simulink model "SingleStreamSSR"  (R2020a)
settings: Solver=VariableStepAuto  StartTime=0.0  StopTime=4096  RelTol=1e-3
PreLoadFcn:
  | xmcCheckSlxPath(bdroot)
  | SSR4_init
undefined symbols (not defined in the file): FIR_MultiKernel_cin, FIR_MultiKernel_cincout, FIR_MultiKernel_cout, N, SHIFT_ACC, SingleStream, Taps, xc7vx485tffg1157
libraries: ModelComposer x37, dspsrcs4 x1, simulink x1
(part 2 of 3)

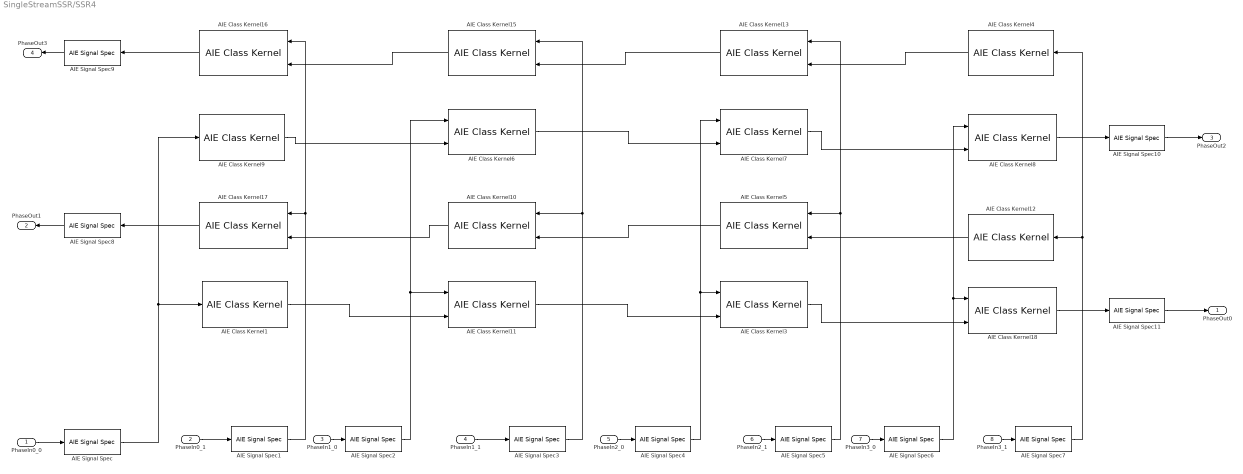
== system SingleStreamSSR/SSR4 ==
  PhaseIn0_0 : Inport
  PhaseIn0_1 : Inport  Port=2
  PhaseIn1_0 : Inport  Port=3
  PhaseIn1_1 : Inport  Port=4
  PhaseIn2_0 : Inport  Port=5
  PhaseIn2_1 : Inport  Port=6
  PhaseIn3_0 : Inport  Port=7
  PhaseIn3_1 : Inport  Port=8
  AIE Class Kernel1 : ModelComposer/AIE Class Kernel  KernelAllAttrs=|  PortNames={'sin'; 'cout'}  PortSerializedTypes={'{P{Tinput_stream{1{t{Scint16}}}}}'; '{P{Toutput_stream{1{t{Scacc48_t}}}}}'}  PortWindowSizes={0.000000000000000000e+00; 0.000000000000000000e+00}  PortWindowMargins={0.000000000000000000e+00; 0.000000000000000000e+00}  PortSynchronicities={'auto'; 'auto'}  PortSignalSizes={0.000000000000000000e+00; 4.000000000000000000e+00}  ClassTemplateSpecKind=implicit  ClassTemplateParamNames={'NSamples'; 'ShiftAcc'}  ClassTemplateParamKinds={'nontype'; 'nontype'}  ClassTemplateParamTypes={'int'; 'int'}  ClassTemplateParamValues={'512', '15'}  ClassCtorParamNames={'taps'; 'Delay'}  ClassCtorParamSerializedTypes={'{R{Q1{C{Scint16}8}}}'; '{Q1{Bi32}}'}  ClassCtorParamValues={'[-54-21i -121-233i 102-525i 237-96i 8773-2748i 1454+497i 342+439i 14+121i]', '0'}  ClassIndex=1  ClassCtorIndex=1  ClassTabVisible=on  ClassTemplateParamsVisible=on  ClassCtorDeclVisible=on  ClassCtorParamsVisible=on  FunctionTabVisible=on  FunctionDecl=|  PortAttrs={ 'input', 'sin', 'input_stream_cint16 *', '', '', '', ''; 'output', 'cout', 'output_stream< cacc48_t > *', '', '', '', 'N' }  PortAttrsEnables={'off', 'off', 'off', 'off', 'off', 'off', 'off';'off', 'off', 'off', 'off', 'off', 'off', 'on'}  SampleTime=-1  ClassDeclTypeOptions=|  ClassDecl=|  ClassTemplateParams={ 'NSamples', 'int', 'BURST_LENGTH'; 'ShiftAcc', 'int', 'SHIFT_ACC' }  ClassTemplateParamsEnables={'off', 'off', 'on';'off', 'off', 'on'}  ClassCtorDeclTypeOptions=C[1 1]@t70@FIR_MultiKernel_cout(cint16 const ( & taps ) [ 8 ], int32 const Delay)  ClassCtorDecl=FIR_MultiKernel_cout(cint16 const ( & taps ) [ 8 ], int32 const Delay)  ClassCtorParams={ 'taps', 'cint16 const ( &) [ 8 ]', 'phi_0'; 'Delay', 'int32 const', '0' }  KernelHeaderFile=FirSingleStream.h  KernelClassName=SingleStream::FIR_MultiKernel_cout  KernelFunction=filter  KernelSourceFile=FirSingleStream.cpp  KernelSearchPaths={'$SRC', '$SRC/aie_kernels'}  PreProcOptions={}  CoreRuntimeRatio=0.9  KernelLocSpec=on  ColRowLocation=LOCATION_2_0  blockJsonConstraints="[{\"type\":\"constraint\",\"constraintType\":\"coreUtilization\",\"sid\":\"386\",\"lhs\":{\"type\":\"runtimeRatio\",\"args\":{\"type\":\"kernel\",\"name\":\"SingleStreamSSR/SSR4/AIE Class Kernel1\",\"sid\":\"386\"}},\"rhs\":{\"type\":\"evaluable\",\"expr\":\"0.9\",\"value\":0.9},\"equality\":true},{\"type\":\"constraint\",\"constraintType\":\"location_kernel\",\"sid\":\"386\",\"lhs\":{\"type\":\"location\",\"templParam\":\"kernel\",\"args\":{\"type\":\"kernel\",\"name\":\"SingleStreamSSR/SSR4/AIE Class Kernel1\",\"sid\":\"386\"}},\"rhs\":{\"type\":\"tile\",\"args\":[{\"type\":\"evaluable\",\"expr\":\"25\",\"value\":25},{\"type\":\"evaluable\",\"expr\":\"0\",\"value\":0}]},\"equality\":true}]"  deprecateConstraints=1
      KernelAllAttrs=|
      | s[12;12;9;9;19;14;21;23;24;21;12;24;26;26;26;27;28;9;21;23;23;23;24;25;14;19;19;29]@FunctionNameDeclFileNamePortNamesPortTypesPortSerializedTypesPortDirectionsPortWindowSizeEnablesPortWindowMarginEnablesPortSynchronicityEnablesPortSignalSizeEnablesFunctionDeclFunctionTemplateSpecKindFunctionTemplateParamNamesFunctionTemplateParamKindsFunctionTemplateParamTypesFunctionTemplateParamValuesFunctionTemplateParamEnablesClassDeclClassTemplateSpecKindClassTemplateParamNamesClassTemplateParamKindsClassTemplateParamTypesClassTemplateParamValuesClassTemplateParamEnablesClassCtorDeclsClassCtorParamNamesClassCtorParamTypesClassCtorParamSerializedTypes[1 1]@C[28 1]@t6@filtert42@../../../src/aie_kernels/FirSingleStream.hC[2 1]@t3@sint4@coutC[2 1]@t21@input_stream_cint16 *t27@output_stream< cacc48_t > *C[2 1]@t33@{P{Tinput_stream{1{t{Scint16}}}}}t36@{P{Toutput_stream{1{t{Scacc48_t}}}}}C[2 1]@t5@inputt6@outputC[2 1]@l0@l0@C[2 1]@l0@l0@C[2 1]@l0@l0@C[2 1]@l0@l1@t164@namespace SingleStream {
      | template < int NSamples, int ShiftAcc > 
      | void FIR_MultiKernel_cout::
      | filter(input_stream_cint16 * sin, output_stream< cacc48_t > * cout);
      | }t4@nonee[0 1]@e[0 1]@e[0 1]@e[0 1]@e[0 1]@t94@namespace SingleStream {
      | template < int NSamples, int ShiftAcc > class FIR_MultiKernel_cout;
      | }t8@implicitC[2 1]@t8@NSamplest8@ShiftAccC[2 1]@t7@nontypet7@nontypeC[2 1]@t3@intt3@intC[2 1]@nnC[2 1]@l1@l1@C[1 1]@t70@FIR_MultiKernel_cout(cint16 const ( & taps ) [ 8 ], int32 const Delay)C[1 1]@C[2 1]@t4@tapst5@DelayC[1 1]@C[2 1]@t23@cint16 const ( &) [ 8 ]t11@int32 constC[1 1]@C[2 1]@t20@{R{Q1{C{Scint16}8}}}t10@{Q1{Bi32}}
      FunctionDecl=|
      | namespace SingleStream {
      | template < int NSamples, int ShiftAcc > 
      | void FIR_MultiKernel_cout::
      | filter(input_stream_cint16 * sin, output_stream< cacc48_t > * cout);
      | }
      ClassDeclTypeOptions=|
      | C[1 1]@t94@namespace SingleStream {
      | template < int NSamples, int ShiftAcc > class FIR_MultiKernel_cout;
      | }
      ClassDecl=|
      | namespace SingleStream {
      | template < int NSamples, int ShiftAcc > class FIR_MultiKernel_cout;
      | }
  AIE Class Kernel10 : ModelComposer/AIE Class Kernel  KernelAllAttrs=|  PortNames={'sin'; 'cin'; 'cout'}  PortSerializedTypes={'{P{Tinput_stream{1{t{Scint16}}}}}'; '{P{Tinput_stream{1{t{Scacc48_t}}}}}'; '{P{Toutput_stream{1{t{Scacc48_t}}}}}'}  PortWindowSizes={0.000000000000000000e+00; 0.000000000000000000e+00; 0.000000000000000000e+00}  PortWindowMargins={0.000000000000000000e+00; 0.000000000000000000e+00; 0.000000000000000000e+00}  PortSynchronicities={'auto'; 'auto'; 'auto'}  PortSignalSizes={0.000000000000000000e+00; 0.000000000000000000e+00; 4.000000000000000000e+00}  ClassTemplateSpecKind=implicit  ClassTemplateParamNames={'NSamples'; 'ShiftAcc'}  ClassTemplateParamKinds={'nontype'; 'nontype'}  ClassTemplateParamTypes={'int'; 'int'}  ClassTemplateParamValues={'512', '15'}  ClassCtorParamNames={'taps'; 'Delay'}  ClassCtorParamSerializedTypes={'{R{Q1{C{Scint16}8}}}'; '{Q1{Bi32}}'}  ClassCtorParamValues={'[-54-21i -121-233i 102-525i 237-96i 8773-2748i 1454+497i 342+439i 14+121i]', '0'}  ClassIndex=1  ClassCtorIndex=1  ClassTabVisible=on  ClassTemplateParamsVisible=on  ClassCtorDeclVisible=on  ClassCtorParamsVisible=on  FunctionTabVisible=on  FunctionDecl=|  PortAttrs={ 'input', 'sin', 'input_stream_cint16 *', '', '', '', ''; 'input', 'cin', 'input_stream< cacc48_t > *', '', '', '', ''; 'output', 'cout', 'output_stream< cacc48_t > *', '', '', '', 'N' }  PortAttrsEnables={'off', 'off', 'off', 'off', 'off', 'off', 'off';'off', 'off', 'off', 'off', 'off', 'off', 'off';'off', 'off', 'off', 'off', 'off', 'off', 'on'}  SampleTime=-1  ClassDeclTypeOptions=|  ClassDecl=|  ClassTemplateParams={ 'NSamples', 'int', 'BURST_LENGTH'; 'ShiftAcc', 'int', 'SHIFT_ACC' }  ClassTemplateParamsEnables={'off', 'off', 'on';'off', 'off', 'on'}  ClassCtorDeclTypeOptions=C[1 1]@t73@FIR_MultiKernel_cincout(cint16 const ( & taps ) [ 8 ], int32 const Delay)  ClassCtorDecl=FIR_MultiKernel_cincout(cint16 const ( & taps ) [ 8 ], int32 const Delay)  ClassCtorParams={ 'taps', 'cint16 const ( &) [ 8 ]', 'phi_0'; 'Delay', 'int32 const', '0' }  KernelHeaderFile=FirSingleStream.h  KernelClassName=SingleStream::FIR_MultiKernel_cincout  KernelFunction=filter  KernelSourceFile=FirSingleStream.cpp  KernelSearchPaths={'$SRC', '$SRC/aie_kernels'}  PreProcOptions={}  CoreRuntimeRatio=0.9  KernelLocSpec=off  ColRowLocation=[25 0]  blockJsonConstraints="{\"type\":\"constraint\",\"constraintType\":\"coreUtilization\",\"sid\":\"396\",\"lhs\":{\"type\":\"runtimeRatio\",\"args\":{\"type\":\"kernel\",\"name\":\"SingleStreamSSR/SSR4/AIE Class Kernel10\",\"sid\":\"396\"}},\"rhs\":{\"type\":\"evaluable\",\"expr\":\"0.9\",\"value\":0.9},\"equality\":true}"  deprecateConstraints=1
      KernelAllAttrs=|
      | s[12;12;9;9;19;14;21;23;24;21;12;24;26;26;26;27;28;9;21;23;23;23;24;25;14;19;19;29]@FunctionNameDeclFileNamePortNamesPortTypesPortSerializedTypesPortDirectionsPortWindowSizeEnablesPortWindowMarginEnablesPortSynchronicityEnablesPortSignalSizeEnablesFunctionDeclFunctionTemplateSpecKindFunctionTemplateParamNamesFunctionTemplateParamKindsFunctionTemplateParamTypesFunctionTemplateParamValuesFunctionTemplateParamEnablesClassDeclClassTemplateSpecKindClassTemplateParamNamesClassTemplateParamKindsClassTemplateParamTypesClassTemplateParamValuesClassTemplateParamEnablesClassCtorDeclsClassCtorParamNamesClassCtorParamTypesClassCtorParamSerializedTypes[1 1]@C[28 1]@t6@filtert42@../../../src/aie_kernels/FirSingleStream.hC[3 1]@t3@sint3@cint4@coutC[3 1]@t21@input_stream_cint16 *t26@input_stream< cacc48_t > *t27@output_stream< cacc48_t > *C[3 1]@t33@{P{Tinput_stream{1{t{Scint16}}}}}t35@{P{Tinput_stream{1{t{Scacc48_t}}}}}t36@{P{Toutput_stream{1{t{Scacc48_t}}}}}C[3 1]@t5@inputt5@inputt6@outputC[3 1]@l0@l0@l0@C[3 1]@l0@l0@l0@C[3 1]@l0@l0@l0@C[3 1]@l0@l0@l1@t199@namespace SingleStream {
      | template < int NSamples, int ShiftAcc > 
      | void FIR_MultiKernel_cincout::
      | filter(input_stream_cint16 * sin, input_stream< cacc48_t > * cin, output_stream< cacc48_t > * cout);
      | }t4@nonee[0 1]@e[0 1]@e[0 1]@e[0 1]@e[0 1]@t97@namespace SingleStream {
      | template < int NSamples, int ShiftAcc > class FIR_MultiKernel_cincout;
      | }t8@implicitC[2 1]@t8@NSamplest8@ShiftAccC[2 1]@t7@nontypet7@nontypeC[2 1]@t3@intt3@intC[2 1]@nnC[2 1]@l1@l1@C[1 1]@t73@FIR_MultiKernel_cincout(cint16 const ( & taps ) [ 8 ], int32 const Delay)C[1 1]@C[2 1]@t4@tapst5@DelayC[1 1]@C[2 1]@t23@cint16 const ( &) [ 8 ]t11@int32 constC[1 1]@C[2 1]@t20@{R{Q1{C{Scint16}8}}}t10@{Q1{Bi32}}
      FunctionDecl=|
      | namespace SingleStream {
      | template < int NSamples, int ShiftAcc > 
      | void FIR_MultiKernel_cincout::
      | filter(input_stream_cint16 * sin, input_stream< cacc48_t > * cin, output_stream< cacc48_t > * cout);
      | }
      ClassDeclTypeOptions=|
      | C[1 1]@t97@namespace SingleStream {
      | template < int NSamples, int ShiftAcc > class FIR_MultiKernel_cincout;
      | }
      ClassDecl=|
      | namespace SingleStream {
      | template < int NSamples, int ShiftAcc > class FIR_MultiKernel_cincout;
      | }
  AIE Class Kernel11 : ModelComposer/AIE Class Kernel  KernelAllAttrs=|  PortNames={'sin'; 'cin'; 'cout'}  PortSerializedTypes={'{P{Tinput_stream{1{t{Scint16}}}}}'; '{P{Tinput_stream{1{t{Scacc48_t}}}}}'; '{P{Toutput_stream{1{t{Scacc48_t}}}}}'}  PortWindowSizes={0.000000000000000000e+00; 0.000000000000000000e+00; 0.000000000000000000e+00}  PortWindowMargins={0.000000000000000000e+00; 0.000000000000000000e+00; 0.000000000000000000e+00}  PortSynchronicities={'auto'; 'auto'; 'auto'}  PortSignalSizes={0.000000000000000000e+00; 0.000000000000000000e+00; 4.000000000000000000e+00}  ClassTemplateSpecKind=implicit  ClassTemplateParamNames={'NSamples'; 'ShiftAcc'}  ClassTemplateParamKinds={'nontype'; 'nontype'}  ClassTemplateParamTypes={'int'; 'int'}  ClassTemplateParamValues={'512', '15'}  ClassCtorParamNames={'taps'; 'Delay'}  ClassCtorParamSerializedTypes={'{R{Q1{C{Scint16}8}}}'; '{Q1{Bi32}}'}  ClassCtorParamValues={'[-83+21i -160-111i 237+54i 248+2878i 4086-5221i 1183-239i 146+91i -21-26i]', '0'}  ClassIndex=1  ClassCtorIndex=1  ClassTabVisible=on  ClassTemplateParamsVisible=on  ClassCtorDeclVisible=on  ClassCtorParamsVisible=on  FunctionTabVisible=on  FunctionDecl=|  PortAttrs={ 'input', 'sin', 'input_stream_cint16 *', '', '', '', ''; 'input', 'cin', 'input_stream< cacc48_t > *', '', '', '', ''; 'output', 'cout', 'output_stream< cacc48_t > *', '', '', '', 'N' }  PortAttrsEnables={'off', 'off', 'off', 'off', 'off', 'off', 'off';'off', 'off', 'off', 'off', 'off', 'off', 'off';'off', 'off', 'off', 'off', 'off', 'off', 'on'}  SampleTime=-1  ClassDeclTypeOptions=|  ClassDecl=|  ClassTemplateParams={ 'NSamples', 'int', 'BURST_LENGTH'; 'ShiftAcc', 'int', 'SHIFT_ACC' }  ClassTemplateParamsEnables={'off', 'off', 'on';'off', 'off', 'on'}  ClassCtorDeclTypeOptions=C[1 1]@t73@FIR_MultiKernel_cincout(cint16 const ( & taps ) [ 8 ], int32 const Delay)  ClassCtorDecl=FIR_MultiKernel_cincout(cint16 const ( & taps ) [ 8 ], int32 const Delay)  ClassCtorParams={ 'taps', 'cint16 const ( &) [ 8 ]', 'phi_1'; 'Delay', 'int32 const', '0' }  KernelHeaderFile=FirSingleStream.h  KernelClassName=SingleStream::FIR_MultiKernel_cincout  KernelFunction=filter  KernelSourceFile=FirSingleStream.cpp  KernelSearchPaths={'$SRC', '$SRC/aie_kernels'}  PreProcOptions={}  CoreRuntimeRatio=0.9  KernelLocSpec=off  ColRowLocation=[25 0]  blockJsonConstraints="{\"type\":\"constraint\",\"constraintType\":\"coreUtilization\",\"sid\":\"399\",\"lhs\":{\"type\":\"runtimeRatio\",\"args\":{\"type\":\"kernel\",\"name\":\"SingleStreamSSR/SSR4/AIE Class Kernel11\",\"sid\":\"399\"}},\"rhs\":{\"type\":\"evaluable\",\"expr\":\"0.9\",\"value\":0.9},\"equality\":true}"  deprecateConstraints=1
      KernelAllAttrs=|
      | s[12;12;9;9;19;14;21;23;24;21;12;24;26;26;26;27;28;9;21;23;23;23;24;25;14;19;19;29]@FunctionNameDeclFileNamePortNamesPortTypesPortSerializedTypesPortDirectionsPortWindowSizeEnablesPortWindowMarginEnablesPortSynchronicityEnablesPortSignalSizeEnablesFunctionDeclFunctionTemplateSpecKindFunctionTemplateParamNamesFunctionTemplateParamKindsFunctionTemplateParamTypesFunctionTemplateParamValuesFunctionTemplateParamEnablesClassDeclClassTemplateSpecKindClassTemplateParamNamesClassTemplateParamKindsClassTemplateParamTypesClassTemplateParamValuesClassTemplateParamEnablesClassCtorDeclsClassCtorParamNamesClassCtorParamTypesClassCtorParamSerializedTypes[1 1]@C[28 1]@t6@filtert42@../../../src/aie_kernels/FirSingleStream.hC[3 1]@t3@sint3@cint4@coutC[3 1]@t21@input_stream_cint16 *t26@input_stream< cacc48_t > *t27@output_stream< cacc48_t > *C[3 1]@t33@{P{Tinput_stream{1{t{Scint16}}}}}t35@{P{Tinput_stream{1{t{Scacc48_t}}}}}t36@{P{Toutput_stream{1{t{Scacc48_t}}}}}C[3 1]@t5@inputt5@inputt6@outputC[3 1]@l0@l0@l0@C[3 1]@l0@l0@l0@C[3 1]@l0@l0@l0@C[3 1]@l0@l0@l1@t199@namespace SingleStream {
      | template < int NSamples, int ShiftAcc > 
      | void FIR_MultiKernel_cincout::
      | filter(input_stream_cint16 * sin, input_stream< cacc48_t > * cin, output_stream< cacc48_t > * cout);
      | }t4@nonee[0 1]@e[0 1]@e[0 1]@e[0 1]@e[0 1]@t97@namespace SingleStream {
      | template < int NSamples, int ShiftAcc > class FIR_MultiKernel_cincout;
      | }t8@implicitC[2 1]@t8@NSamplest8@ShiftAccC[2 1]@t7@nontypet7@nontypeC[2 1]@t3@intt3@intC[2 1]@nnC[2 1]@l1@l1@C[1 1]@t73@FIR_MultiKernel_cincout(cint16 const ( & taps ) [ 8 ], int32 const Delay)C[1 1]@C[2 1]@t4@tapst5@DelayC[1 1]@C[2 1]@t23@cint16 const ( &) [ 8 ]t11@int32 constC[1 1]@C[2 1]@t20@{R{Q1{C{Scint16}8}}}t10@{Q1{Bi32}}
      FunctionDecl=|
      | namespace SingleStream {
      | template < int NSamples, int ShiftAcc > 
      | void FIR_MultiKernel_cincout::
      | filter(input_stream_cint16 * sin, input_stream< cacc48_t > * cin, output_stream< cacc48_t > * cout);
      | }
      ClassDeclTypeOptions=|
      | C[1 1]@t97@namespace SingleStream {
      | template < int NSamples, int ShiftAcc > class FIR_MultiKernel_cincout;
      | }
      ClassDecl=|
      | namespace SingleStream {
      | template < int NSamples, int ShiftAcc > class FIR_MultiKernel_cincout;
      | }
  AIE Class Kernel12 : ModelComposer/AIE Class Kernel  KernelAllAttrs=|  PortNames={'sin'; 'cout'}  PortSerializedTypes={'{P{Tinput_stream{1{t{Scint16}}}}}'; '{P{Toutput_stream{1{t{Scacc48_t}}}}}'}  PortWindowSizes={0.000000000000000000e+00; 0.000000000000000000e+00}  PortWindowMargins={0.000000000000000000e+00; 0.000000000000000000e+00}  PortSynchronicities={'auto'; 'auto'}  PortSignalSizes={0.000000000000000000e+00; 4.000000000000000000e+00}  ClassTemplateSpecKind=implicit  ClassTemplateParamNames={'NSamples'; 'ShiftAcc'}  ClassTemplateParamKinds={'nontype'; 'nontype'}  ClassTemplateParamTypes={'int'; 'int'}  ClassTemplateParamValues={'512', '15'}  ClassCtorParamNames={'taps'; 'Delay'}  ClassCtorParamSerializedTypes={'{R{Q1{C{Scint16}8}}}'; '{Q1{Bi32}}'}  ClassCtorParamValues={'[-21+26i 146-91i 1183+239i 4086+5221i 248-2878i 237-54i -160+111i -83-21i]', '0'}  ClassIndex=1  ClassCtorIndex=1  ClassTabVisible=on  ClassTemplateParamsVisible=on  ClassCtorDeclVisible=on  ClassCtorParamsVisible=on  FunctionTabVisible=on  FunctionDecl=|  PortAttrs={ 'input', 'sin', 'input_stream_cint16 *', '', '', '', ''; 'output', 'cout', 'output_stream< cacc48_t > *', '', '', '', 'N' }  PortAttrsEnables={'off', 'off', 'off', 'off', 'off', 'off', 'off';'off', 'off', 'off', 'off', 'off', 'off', 'on'}  SampleTime=-1  ClassDeclTypeOptions=|  ClassDecl=|  ClassTemplateParams={ 'NSamples', 'int', 'BURST_LENGTH'; 'ShiftAcc', 'int', 'SHIFT_ACC' }  ClassTemplateParamsEnables={'off', 'off', 'on';'off', 'off', 'on'}  ClassCtorDeclTypeOptions=C[1 1]@t70@FIR_MultiKernel_cout(cint16 const ( & taps ) [ 8 ], int32 const Delay)  ClassCtorDecl=FIR_MultiKernel_cout(cint16 const ( & taps ) [ 8 ], int32 const Delay)  ClassCtorParams={ 'taps', 'cint16 const ( &) [ 8 ]', 'phi_2'; 'Delay', 'int32 const', '0' }  KernelHeaderFile=FirSingleStream.h  KernelClassName=SingleStream::FIR_MultiKernel_cout  KernelFunction=filter  KernelSourceFile=FirSingleStream.cpp  KernelSearchPaths={'$SRC', '$SRC/aie_kernels'}  PreProcOptions={}  CoreRuntimeRatio=0.9  KernelLocSpec=on  ColRowLocation=LOCATION_2_0  blockJsonConstraints="[{\"type\":\"constraint\",\"constraintType\":\"coreUtilization\",\"sid\":\"388\",\"lhs\":{\"type\":\"runtimeRatio\",\"args\":{\"type\":\"kernel\",\"name\":\"SingleStreamSSR/SSR4/AIE Class Kernel12\",\"sid\":\"388\"}},\"rhs\":{\"type\":\"evaluable\",\"expr\":\"0.9\",\"value\":0.9},\"equality\":true},{\"type\":\"constraint\",\"constraintType\":\"location_kernel\",\"sid\":\"388\",\"lhs\":{\"type\":\"location\",\"templParam\":\"kernel\",\"args\":{\"type\":\"kernel\",\"name\":\"SingleStreamSSR/SSR4/AIE Class Kernel12\",\"sid\":\"388\"}},\"rhs\":{\"type\":\"tile\",\"args\":[{\"type\":\"evaluable\",\"expr\":\"28\",\"value\":28},{\"type\":\"evaluable\",\"expr\":\"1\",\"value\":1}]},\"equality\":true}]"  deprecateConstraints=1
      KernelAllAttrs=|
      | s[12;12;9;9;19;14;21;23;24;21;12;24;26;26;26;27;28;9;21;23;23;23;24;25;14;19;19;29]@FunctionNameDeclFileNamePortNamesPortTypesPortSerializedTypesPortDirectionsPortWindowSizeEnablesPortWindowMarginEnablesPortSynchronicityEnablesPortSignalSizeEnablesFunctionDeclFunctionTemplateSpecKindFunctionTemplateParamNamesFunctionTemplateParamKindsFunctionTemplateParamTypesFunctionTemplateParamValuesFunctionTemplateParamEnablesClassDeclClassTemplateSpecKindClassTemplateParamNamesClassTemplateParamKindsClassTemplateParamTypesClassTemplateParamValuesClassTemplateParamEnablesClassCtorDeclsClassCtorParamNamesClassCtorParamTypesClassCtorParamSerializedTypes[1 1]@C[28 1]@t6@filtert42@../../../src/aie_kernels/FirSingleStream.hC[2 1]@t3@sint4@coutC[2 1]@t21@input_stream_cint16 *t27@output_stream< cacc48_t > *C[2 1]@t33@{P{Tinput_stream{1{t{Scint16}}}}}t36@{P{Toutput_stream{1{t{Scacc48_t}}}}}C[2 1]@t5@inputt6@outputC[2 1]@l0@l0@C[2 1]@l0@l0@C[2 1]@l0@l0@C[2 1]@l0@l1@t164@namespace SingleStream {
      | template < int NSamples, int ShiftAcc > 
      | void FIR_MultiKernel_cout::
      | filter(input_stream_cint16 * sin, output_stream< cacc48_t > * cout);
      | }t4@nonee[0 1]@e[0 1]@e[0 1]@e[0 1]@e[0 1]@t94@namespace SingleStream {
      | template < int NSamples, int ShiftAcc > class FIR_MultiKernel_cout;
      | }t8@implicitC[2 1]@t8@NSamplest8@ShiftAccC[2 1]@t7@nontypet7@nontypeC[2 1]@t3@intt3@intC[2 1]@nnC[2 1]@l1@l1@C[1 1]@t70@FIR_MultiKernel_cout(cint16 const ( & taps ) [ 8 ], int32 const Delay)C[1 1]@C[2 1]@t4@tapst5@DelayC[1 1]@C[2 1]@t23@cint16 const ( &) [ 8 ]t11@int32 constC[1 1]@C[2 1]@t20@{R{Q1{C{Scint16}8}}}t10@{Q1{Bi32}}
      FunctionDecl=|
      | namespace SingleStream {
      | template < int NSamples, int ShiftAcc > 
      | void FIR_MultiKernel_cout::
      | filter(input_stream_cint16 * sin, output_stream< cacc48_t > * cout);
      | }
      ClassDeclTypeOptions=|
      | C[1 1]@t94@namespace SingleStream {
      | template < int NSamples, int ShiftAcc > class FIR_MultiKernel_cout;
      | }
      ClassDecl=|
      | namespace SingleStream {
      | template < int NSamples, int ShiftAcc > class FIR_MultiKernel_cout;
      | }
  AIE Class Kernel13 : ModelComposer/AIE Class Kernel  KernelAllAttrs=|  PortNames={'sin'; 'cin'; 'cout'}  PortSerializedTypes={'{P{Tinput_stream{1{t{Scint16}}}}}'; '{P{Tinput_stream{1{t{Scacc48_t}}}}}'; '{P{Toutput_stream{1{t{Scacc48_t}}}}}'}  PortWindowSizes={0.000000000000000000e+00; 0.000000000000000000e+00; 0.000000000000000000e+00}  PortWindowMargins={0.000000000000000000e+00; 0.000000000000000000e+00; 0.000000000000000000e+00}  PortSynchronicities={'auto'; 'auto'; 'auto'}  PortSignalSizes={0.000000000000000000e+00; 0.000000000000000000e+00; 4.000000000000000000e+00}  ClassTemplateSpecKind=implicit  ClassTemplateParamNames={'NSamples'; 'ShiftAcc'}  ClassTemplateParamKinds={'nontype'; 'nontype'}  ClassTemplateParamTypes={'int'; 'int'}  ClassTemplateParamValues={'512', '15'}  ClassCtorParamNames={'taps'; 'Delay'}  ClassCtorParamSerializedTypes={'{R{Q1{C{Scint16}8}}}'; '{Q1{Bi32}}'}  ClassCtorParamValues={'[14-121i 342-439i 1454-497i 8773+2748i 237+96i 102+525i -121+233i -54+21i]', '1'}  ClassIndex=1  ClassCtorIndex=1  ClassTabVisible=on  ClassTemplateParamsVisible=on  ClassCtorDeclVisible=on  ClassCtorParamsVisible=on  FunctionTabVisible=on  FunctionDecl=|  PortAttrs={ 'input', 'sin', 'input_stream_cint16 *', '', '', '', ''; 'input', 'cin', 'input_stream< cacc48_t > *', '', '', '', ''; 'output', 'cout', 'output_stream< cacc48_t > *', '', '', '', 'N' }  PortAttrsEnables={'off', 'off', 'off', 'off', 'off', 'off', 'off';'off', 'off', 'off', 'off', 'off', 'off', 'off';'off', 'off', 'off', 'off', 'off', 'off', 'on'}  SampleTime=-1  ClassDeclTypeOptions=|  ClassDecl=|  ClassTemplateParams={ 'NSamples', 'int', 'BURST_LENGTH'; 'ShiftAcc', 'int', 'SHIFT_ACC' }  ClassTemplateParamsEnables={'off', 'off', 'on';'off', 'off', 'on'}  ClassCtorDeclTypeOptions=C[1 1]@t73@FIR_MultiKernel_cincout(cint16 const ( & taps ) [ 8 ], int32 const Delay)  ClassCtorDecl=FIR_MultiKernel_cincout(cint16 const ( & taps ) [ 8 ], int32 const Delay)  ClassCtorParams={ 'taps', 'cint16 const ( &) [ 8 ]', 'phi_3'; 'Delay', 'int32 const', '1' }  KernelHeaderFile=FirSingleStream.h  KernelClassName=SingleStream::FIR_MultiKernel_cincout  KernelFunction=filter  KernelSourceFile=FirSingleStream.cpp  KernelSearchPaths={'$SRC', '$SRC/aie_kernels'}  PreProcOptions={}  CoreRuntimeRatio=0.9  KernelLocSpec=off  ColRowLocation=[25 0]  blockJsonConstraints="{\"type\":\"constraint\",\"constraintType\":\"coreUtilization\",\"sid\":\"392\",\"lhs\":{\"type\":\"runtimeRatio\",\"args\":{\"type\":\"kernel\",\"name\":\"SingleStreamSSR/SSR4/AIE Class Kernel13\",\"sid\":\"392\"}},\"rhs\":{\"type\":\"evaluable\",\"expr\":\"0.9\",\"value\":0.9},\"equality\":true}"  deprecateConstraints=1
      KernelAllAttrs=|
      | s[12;12;9;9;19;14;21;23;24;21;12;24;26;26;26;27;28;9;21;23;23;23;24;25;14;19;19;29]@FunctionNameDeclFileNamePortNamesPortTypesPortSerializedTypesPortDirectionsPortWindowSizeEnablesPortWindowMarginEnablesPortSynchronicityEnablesPortSignalSizeEnablesFunctionDeclFunctionTemplateSpecKindFunctionTemplateParamNamesFunctionTemplateParamKindsFunctionTemplateParamTypesFunctionTemplateParamValuesFunctionTemplateParamEnablesClassDeclClassTemplateSpecKindClassTemplateParamNamesClassTemplateParamKindsClassTemplateParamTypesClassTemplateParamValuesClassTemplateParamEnablesClassCtorDeclsClassCtorParamNamesClassCtorParamTypesClassCtorParamSerializedTypes[1 1]@C[28 1]@t6@filtert42@../../../src/aie_kernels/FirSingleStream.hC[3 1]@t3@sint3@cint4@coutC[3 1]@t21@input_stream_cint16 *t26@input_stream< cacc48_t > *t27@output_stream< cacc48_t > *C[3 1]@t33@{P{Tinput_stream{1{t{Scint16}}}}}t35@{P{Tinput_stream{1{t{Scacc48_t}}}}}t36@{P{Toutput_stream{1{t{Scacc48_t}}}}}C[3 1]@t5@inputt5@inputt6@outputC[3 1]@l0@l0@l0@C[3 1]@l0@l0@l0@C[3 1]@l0@l0@l0@C[3 1]@l0@l0@l1@t199@namespace SingleStream {
      | template < int NSamples, int ShiftAcc > 
      | void FIR_MultiKernel_cincout::
      | filter(input_stream_cint16 * sin, input_stream< cacc48_t > * cin, output_stream< cacc48_t > * cout);
      | }t4@nonee[0 1]@e[0 1]@e[0 1]@e[0 1]@e[0 1]@t97@namespace SingleStream {
      | template < int NSamples, int ShiftAcc > class FIR_MultiKernel_cincout;
      | }t8@implicitC[2 1]@t8@NSamplest8@ShiftAccC[2 1]@t7@nontypet7@nontypeC[2 1]@t3@intt3@intC[2 1]@nnC[2 1]@l1@l1@C[1 1]@t73@FIR_MultiKernel_cincout(cint16 const ( & taps ) [ 8 ], int32 const Delay)C[1 1]@C[2 1]@t4@tapst5@DelayC[1 1]@C[2 1]@t23@cint16 const ( &) [ 8 ]t11@int32 constC[1 1]@C[2 1]@t20@{R{Q1{C{Scint16}8}}}t10@{Q1{Bi32}}
      FunctionDecl=|
      | namespace SingleStream {
      | template < int NSamples, int ShiftAcc > 
      | void FIR_MultiKernel_cincout::
      | filter(input_stream_cint16 * sin, input_stream< cacc48_t > * cin, output_stream< cacc48_t > * cout);
      | }
      ClassDeclTypeOptions=|
      | C[1 1]@t97@namespace SingleStream {
      | template < int NSamples, int ShiftAcc > class FIR_MultiKernel_cincout;
      | }
      ClassDecl=|
      | namespace SingleStream {
      | template < int NSamples, int ShiftAcc > class FIR_MultiKernel_cincout;
      | }
  AIE Class Kernel15 : ModelComposer/AIE Class Kernel  KernelAllAttrs=|  PortNames={'sin'; 'cin'; 'cout'}  PortSerializedTypes={'{P{Tinput_stream{1{t{Scint16}}}}}'; '{P{Tinput_stream{1{t{Scacc48_t}}}}}'; '{P{Toutput_stream{1{t{Scacc48_t}}}}}'}  PortWindowSizes={0.000000000000000000e+00; 0.000000000000000000e+00; 0.000000000000000000e+00}  PortWindowMargins={0.000000000000000000e+00; 0.000000000000000000e+00; 0.000000000000000000e+00}  PortSynchronicities={'auto'; 'auto'; 'auto'}  PortSignalSizes={0.000000000000000000e+00; 0.000000000000000000e+00; 4.000000000000000000e+00}  ClassTemplateSpecKind=implicit  ClassTemplateParamNames={'NSamples'; 'ShiftAcc'}  ClassTemplateParamKinds={'nontype'; 'nontype'}  ClassTemplateParamTypes={'int'; 'int'}  ClassTemplateParamValues={'512', '15'}  ClassCtorParamNames={'taps'; 'Delay'}  ClassCtorParamSerializedTypes={'{R{Q1{C{Scint16}8}}}'; '{Q1{Bi32}}'}  ClassCtorParamValues={'[-21+26i 146-91i 1183+239i 4086+5221i 248-2878i 237-54i -160+111i -83-21i]', '1'}  ClassIndex=1  ClassCtorIndex=1  ClassTabVisible=on  ClassTemplateParamsVisible=on  ClassCtorDeclVisible=on  ClassCtorParamsVisible=on  FunctionTabVisible=on  FunctionDecl=|  PortAttrs={ 'input', 'sin', 'input_stream_cint16 *', '', '', '', ''; 'input', 'cin', 'input_stream< cacc48_t > *', '', '', '', ''; 'output', 'cout', 'output_stream< cacc48_t > *', '', '', '', 'N' }  PortAttrsEnables={'off', 'off', 'off', 'off', 'off', 'off', 'off';'off', 'off', 'off', 'off', 'off', 'off', 'off';'off', 'off', 'off', 'off', 'off', 'off', 'on'}  SampleTime=-1  ClassDeclTypeOptions=|  ClassDecl=|  ClassTemplateParams={ 'NSamples', 'int', 'BURST_LENGTH'; 'ShiftAcc', 'int', 'SHIFT_ACC' }  ClassTemplateParamsEnables={'off', 'off', 'on';'off', 'off', 'on'}  ClassCtorDeclTypeOptions=C[1 1]@t73@FIR_MultiKernel_cincout(cint16 const ( & taps ) [ 8 ], int32 const Delay)  ClassCtorDecl=FIR_MultiKernel_cincout(cint16 const ( & taps ) [ 8 ], int32 const Delay)  ClassCtorParams={ 'taps', 'cint16 const ( &) [ 8 ]', 'phi_2'; 'Delay', 'int32 const', '1' }  KernelHeaderFile=FirSingleStream.h  KernelClassName=SingleStream::FIR_MultiKernel_cincout  KernelFunction=filter  KernelSourceFile=FirSingleStream.cpp  KernelSearchPaths={'$SRC', '$SRC/aie_kernels'}  PreProcOptions={}  CoreRuntimeRatio=0.9  KernelLocSpec=off  ColRowLocation=[25 0]  blockJsonConstraints="{\"type\":\"constraint\",\"constraintType\":\"coreUtilization\",\"sid\":\"332\",\"lhs\":{\"type\":\"runtimeRatio\",\"args\":{\"type\":\"kernel\",\"name\":\"SingleStreamSSR/SSR4/AIE Class Kernel15\",\"sid\":\"332\"}},\"rhs\":{\"type\":\"evaluable\",\"expr\":\"0.9\",\"value\":0.9},\"equality\":true}"  deprecateConstraints=1
      KernelAllAttrs=|
      | s[12;12;9;9;19;14;21;23;24;21;12;24;26;26;26;27;28;9;21;23;23;23;24;25;14;19;19;29]@FunctionNameDeclFileNamePortNamesPortTypesPortSerializedTypesPortDirectionsPortWindowSizeEnablesPortWindowMarginEnablesPortSynchronicityEnablesPortSignalSizeEnablesFunctionDeclFunctionTemplateSpecKindFunctionTemplateParamNamesFunctionTemplateParamKindsFunctionTemplateParamTypesFunctionTemplateParamValuesFunctionTemplateParamEnablesClassDeclClassTemplateSpecKindClassTemplateParamNamesClassTemplateParamKindsClassTemplateParamTypesClassTemplateParamValuesClassTemplateParamEnablesClassCtorDeclsClassCtorParamNamesClassCtorParamTypesClassCtorParamSerializedTypes[1 1]@C[28 1]@t6@filtert42@../../../src/aie_kernels/FirSingleStream.hC[3 1]@t3@sint3@cint4@coutC[3 1]@t21@input_stream_cint16 *t26@input_stream< cacc48_t > *t27@output_stream< cacc48_t > *C[3 1]@t33@{P{Tinput_stream{1{t{Scint16}}}}}t35@{P{Tinput_stream{1{t{Scacc48_t}}}}}t36@{P{Toutput_stream{1{t{Scacc48_t}}}}}C[3 1]@t5@inputt5@inputt6@outputC[3 1]@l0@l0@l0@C[3 1]@l0@l0@l0@C[3 1]@l0@l0@l0@C[3 1]@l0@l0@l1@t199@namespace SingleStream {
      | template < int NSamples, int ShiftAcc > 
      | void FIR_MultiKernel_cincout::
      | filter(input_stream_cint16 * sin, input_stream< cacc48_t > * cin, output_stream< cacc48_t > * cout);
      | }t4@nonee[0 1]@e[0 1]@e[0 1]@e[0 1]@e[0 1]@t97@namespace SingleStream {
      | template < int NSamples, int ShiftAcc > class FIR_MultiKernel_cincout;
      | }t8@implicitC[2 1]@t8@NSamplest8@ShiftAccC[2 1]@t7@nontypet7@nontypeC[2 1]@t3@intt3@intC[2 1]@nnC[2 1]@l1@l1@C[1 1]@t73@FIR_MultiKernel_cincout(cint16 const ( & taps ) [ 8 ], int32 const Delay)C[1 1]@C[2 1]@t4@tapst5@DelayC[1 1]@C[2 1]@t23@cint16 const ( &) [ 8 ]t11@int32 constC[1 1]@C[2 1]@t20@{R{Q1{C{Scint16}8}}}t10@{Q1{Bi32}}
      FunctionDecl=|
      | namespace SingleStream {
      | template < int NSamples, int ShiftAcc > 
      | void FIR_MultiKernel_cincout::
      | filter(input_stream_cint16 * sin, input_stream< cacc48_t > * cin, output_stream< cacc48_t > * cout);
      | }
      ClassDeclTypeOptions=|
      | C[1 1]@t97@namespace SingleStream {
      | template < int NSamples, int ShiftAcc > class FIR_MultiKernel_cincout;
      | }
      ClassDecl=|
      | namespace SingleStream {
      | template < int NSamples, int ShiftAcc > class FIR_MultiKernel_cincout;
      | }
  AIE Class Kernel16 : ModelComposer/AIE Class Kernel  KernelAllAttrs=|  PortNames={'sin'; 'cin'; 'sout'}  PortSerializedTypes={'{P{Tinput_stream{1{t{Scint16}}}}}'; '{P{Tinput_stream{1{t{Scacc48_t}}}}}'; '{P{Toutput_stream{1{t{Scint16}}}}}'}  PortWindowSizes={0.000000000000000000e+00; 0.000000000000000000e+00; 0.000000000000000000e+00}  PortWindowMargins={0.000000000000000000e+00; 0.000000000000000000e+00; 0.000000000000000000e+00}  PortSynchronicities={'auto'; 'auto'; 'auto'}  PortSignalSizes={0.000000000000000000e+00; 0.000000000000000000e+00; 4.000000000000000000e+00}  ClassTemplateSpecKind=implicit  ClassTemplateParamNames={'NSamples'; 'ShiftAcc'}  ClassTemplateParamKinds={'nontype'; 'nontype'}  ClassTemplateParamTypes={'int'; 'int'}  ClassTemplateParamValues={'512', '15'}  ClassCtorParamNames={'taps'; 'Delay'}  ClassCtorParamSerializedTypes={'{R{Q1{C{Scint16}8}}}'; '{Q1{Bi32}}'}  ClassCtorParamValues={'[-83+21i -160-111i 237+54i 248+2878i 4086-5221i 1183-239i 146+91i -21-26i]', '1'}  ClassIndex=1  ClassCtorIndex=1  ClassTabVisible=on  ClassTemplateParamsVisible=on  ClassCtorDeclVisible=on  ClassCtorParamsVisible=on  FunctionTabVisible=on  FunctionDecl=|  PortAttrs={ 'input', 'sin', 'input_stream_cint16 *', '', '', '', ''; 'input', 'cin', 'input_stream< cacc48_t > *', '', '', '', ''; 'output', 'sout', 'output_stream_cint16 *', '', '', '', 'N' }  PortAttrsEnables={'off', 'off', 'off', 'off', 'off', 'off', 'off';'off', 'off', 'off', 'off', 'off', 'off', 'off';'off', 'off', 'off', 'off', 'off', 'off', 'on'}  SampleTime=-1  ClassDeclTypeOptions=|  ClassDecl=|  ClassTemplateParams={ 'NSamples', 'int', 'BURST_LENGTH'; 'ShiftAcc', 'int', 'SHIFT_ACC' }  ClassTemplateParamsEnables={'off', 'off', 'on';'off', 'off', 'on'}  ClassCtorDeclTypeOptions=C[1 1]@t69@FIR_MultiKernel_cin(cint16 const ( & taps ) [ 8 ], int32 const Delay)  ClassCtorDecl=FIR_MultiKernel_cin(cint16 const ( & taps ) [ 8 ], int32 const Delay)  ClassCtorParams={ 'taps', 'cint16 const ( &) [ 8 ]', 'phi_1'; 'Delay', 'int32 const', '1' }  KernelHeaderFile=FirSingleStream.h  KernelClassName=SingleStream::FIR_MultiKernel_cin  KernelFunction=filter  KernelSourceFile=FirSingleStream.cpp  KernelSearchPaths={'$SRC', '$SRC/aie_kernels'}  PreProcOptions={}  CoreRuntimeRatio=0.9  KernelLocSpec=off  ColRowLocation=[25 0]  blockJsonConstraints="{\"type\":\"constraint\",\"constraintType\":\"coreUtilization\",\"sid\":\"364\",\"lhs\":{\"type\":\"runtimeRatio\",\"args\":{\"type\":\"kernel\",\"name\":\"SingleStreamSSR/SSR4/AIE Class Kernel16\",\"sid\":\"364\"}},\"rhs\":{\"type\":\"evaluable\",\"expr\":\"0.9\",\"value\":0.9},\"equality\":true}"  deprecateConstraints=1
      KernelAllAttrs=|
      | s[12;12;9;9;19;14;21;23;24;21;12;24;26;26;26;27;28;9;21;23;23;23;24;25;14;19;19;29]@FunctionNameDeclFileNamePortNamesPortTypesPortSerializedTypesPortDirectionsPortWindowSizeEnablesPortWindowMarginEnablesPortSynchronicityEnablesPortSignalSizeEnablesFunctionDeclFunctionTemplateSpecKindFunctionTemplateParamNamesFunctionTemplateParamKindsFunctionTemplateParamTypesFunctionTemplateParamValuesFunctionTemplateParamEnablesClassDeclClassTemplateSpecKindClassTemplateParamNamesClassTemplateParamKindsClassTemplateParamTypesClassTemplateParamValuesClassTemplateParamEnablesClassCtorDeclsClassCtorParamNamesClassCtorParamTypesClassCtorParamSerializedTypes[1 1]@C[28 1]@t6@filtert42@../../../src/aie_kernels/FirSingleStream.hC[3 1]@t3@sint3@cint4@soutC[3 1]@t21@input_stream_cint16 *t26@input_stream< cacc48_t > *t22@output_stream_cint16 *C[3 1]@t33@{P{Tinput_stream{1{t{Scint16}}}}}t35@{P{Tinput_stream{1{t{Scacc48_t}}}}}t34@{P{Toutput_stream{1{t{Scint16}}}}}C[3 1]@t5@inputt5@inputt6@outputC[3 1]@l0@l0@l0@C[3 1]@l0@l0@l0@C[3 1]@l0@l0@l0@C[3 1]@l0@l0@l1@t190@namespace SingleStream {
      | template < int NSamples, int ShiftAcc > 
      | void FIR_MultiKernel_cin::
      | filter(input_stream_cint16 * sin, input_stream< cacc48_t > * cin, output_stream_cint16 * sout);
      | }t4@nonee[0 1]@e[0 1]@e[0 1]@e[0 1]@e[0 1]@t93@namespace SingleStream {
      | template < int NSamples, int ShiftAcc > class FIR_MultiKernel_cin;
      | }t8@implicitC[2 1]@t8@NSamplest8@ShiftAccC[2 1]@t7@nontypet7@nontypeC[2 1]@t3@intt3@intC[2 1]@nnC[2 1]@l1@l1@C[1 1]@t69@FIR_MultiKernel_cin(cint16 const ( & taps ) [ 8 ], int32 const Delay)C[1 1]@C[2 1]@t4@tapst5@DelayC[1 1]@C[2 1]@t23@cint16 const ( &) [ 8 ]t11@int32 constC[1 1]@C[2 1]@t20@{R{Q1{C{Scint16}8}}}t10@{Q1{Bi32}}
      FunctionDecl=|
      | namespace SingleStream {
      | template < int NSamples, int ShiftAcc > 
      | void FIR_MultiKernel_cin::
      | filter(input_stream_cint16 * sin, input_stream< cacc48_t > * cin, output_stream_cint16 * sout);
      | }
      ClassDeclTypeOptions=|
      | C[1 1]@t93@namespace SingleStream {
      | template < int NSamples, int ShiftAcc > class FIR_MultiKernel_cin;
      | }
      ClassDecl=|
      | namespace SingleStream {
      | template < int NSamples, int ShiftAcc > class FIR_MultiKernel_cin;
      | }
  AIE Class Kernel17 : ModelComposer/AIE Class Kernel  KernelAllAttrs=|  PortNames={'sin'; 'cin'; 'sout'}  PortSerializedTypes={'{P{Tinput_stream{1{t{Scint16}}}}}'; '{P{Tinput_stream{1{t{Scacc48_t}}}}}'; '{P{Toutput_stream{1{t{Scint16}}}}}'}  PortWindowSizes={0.000000000000000000e+00; 0.000000000000000000e+00; 0.000000000000000000e+00}  PortWindowMargins={0.000000000000000000e+00; 0.000000000000000000e+00; 0.000000000000000000e+00}  PortSynchronicities={'auto'; 'auto'; 'auto'}  PortSignalSizes={0.000000000000000000e+00; 0.000000000000000000e+00; 4.000000000000000000e+00}  ClassTemplateSpecKind=implicit  ClassTemplateParamNames={'NSamples'; 'ShiftAcc'}  ClassTemplateParamKinds={'nontype'; 'nontype'}  ClassTemplateParamTypes={'int'; 'int'}  ClassTemplateParamValues={'512', '15'}  ClassCtorParamNames={'taps'; 'Delay'}  ClassCtorParamSerializedTypes={'{R{Q1{C{Scint16}8}}}'; '{Q1{Bi32}}'}  ClassCtorParamValues={'[14-121i 342-439i 1454-497i 8773+2748i 237+96i 102+525i -121+233i -54+21i]', '1'}  ClassIndex=1  ClassCtorIndex=1  ClassTabVisible=on  ClassTemplateParamsVisible=on  ClassCtorDeclVisible=on  ClassCtorParamsVisible=on  FunctionTabVisible=on  FunctionDecl=|  PortAttrs={ 'input', 'sin', 'input_stream_cint16 *', '', '', '', ''; 'input', 'cin', 'input_stream< cacc48_t > *', '', '', '', ''; 'output', 'sout', 'output_stream_cint16 *', '', '', '', 'N' }  PortAttrsEnables={'off', 'off', 'off', 'off', 'off', 'off', 'off';'off', 'off', 'off', 'off', 'off', 'off', 'off';'off', 'off', 'off', 'off', 'off', 'off', 'on'}  SampleTime=-1  ClassDeclTypeOptions=|  ClassDecl=|  ClassTemplateParams={ 'NSamples', 'int', 'BURST_LENGTH'; 'ShiftAcc', 'int', 'SHIFT_ACC' }  ClassTemplateParamsEnables={'off', 'off', 'on';'off', 'off', 'on'}  ClassCtorDeclTypeOptions=C[1 1]@t69@FIR_MultiKernel_cin(cint16 const ( & taps ) [ 8 ], int32 const Delay)  ClassCtorDecl=FIR_MultiKernel_cin(cint16 const ( & taps ) [ 8 ], int32 const Delay)  ClassCtorParams={ 'taps', 'cint16 const ( &) [ 8 ]', 'phi_3'; 'Delay', 'int32 const', '1' }  KernelHeaderFile=FirSingleStream.h  KernelClassName=SingleStream::FIR_MultiKernel_cin  KernelFunction=filter  KernelSourceFile=FirSingleStream.cpp  KernelSearchPaths={'$SRC', '$SRC/aie_kernels'}  PreProcOptions={}  CoreRuntimeRatio=0.9  KernelLocSpec=off  ColRowLocation=[25 0]  blockJsonConstraints="{\"type\":\"constraint\",\"constraintType\":\"coreUtilization\",\"sid\":\"383\",\"lhs\":{\"type\":\"runtimeRatio\",\"args\":{\"type\":\"kernel\",\"name\":\"SingleStreamSSR/SSR4/AIE Class Kernel17\",\"sid\":\"383\"}},\"rhs\":{\"type\":\"evaluable\",\"expr\":\"0.9\",\"value\":0.9},\"equality\":true}"  deprecateConstraints=1
      KernelAllAttrs=|
      | s[12;12;9;9;19;14;21;23;24;21;12;24;26;26;26;27;28;9;21;23;23;23;24;25;14;19;19;29]@FunctionNameDeclFileNamePortNamesPortTypesPortSerializedTypesPortDirectionsPortWindowSizeEnablesPortWindowMarginEnablesPortSynchronicityEnablesPortSignalSizeEnablesFunctionDeclFunctionTemplateSpecKindFunctionTemplateParamNamesFunctionTemplateParamKindsFunctionTemplateParamTypesFunctionTemplateParamValuesFunctionTemplateParamEnablesClassDeclClassTemplateSpecKindClassTemplateParamNamesClassTemplateParamKindsClassTemplateParamTypesClassTemplateParamValuesClassTemplateParamEnablesClassCtorDeclsClassCtorParamNamesClassCtorParamTypesClassCtorParamSerializedTypes[1 1]@C[28 1]@t6@filtert42@../../../src/aie_kernels/FirSingleStream.hC[3 1]@t3@sint3@cint4@soutC[3 1]@t21@input_stream_cint16 *t26@input_stream< cacc48_t > *t22@output_stream_cint16 *C[3 1]@t33@{P{Tinput_stream{1{t{Scint16}}}}}t35@{P{Tinput_stream{1{t{Scacc48_t}}}}}t34@{P{Toutput_stream{1{t{Scint16}}}}}C[3 1]@t5@inputt5@inputt6@outputC[3 1]@l0@l0@l0@C[3 1]@l0@l0@l0@C[3 1]@l0@l0@l0@C[3 1]@l0@l0@l1@t190@namespace SingleStream {
      | template < int NSamples, int ShiftAcc > 
      | void FIR_MultiKernel_cin::
      | filter(input_stream_cint16 * sin, input_stream< cacc48_t > * cin, output_stream_cint16 * sout);
      | }t4@nonee[0 1]@e[0 1]@e[0 1]@e[0 1]@e[0 1]@t93@namespace SingleStream {
      | template < int NSamples, int ShiftAcc > class FIR_MultiKernel_cin;
      | }t8@implicitC[2 1]@t8@NSamplest8@ShiftAccC[2 1]@t7@nontypet7@nontypeC[2 1]@t3@intt3@intC[2 1]@nnC[2 1]@l1@l1@C[1 1]@t69@FIR_MultiKernel_cin(cint16 const ( & taps ) [ 8 ], int32 const Delay)C[1 1]@C[2 1]@t4@tapst5@DelayC[1 1]@C[2 1]@t23@cint16 const ( &) [ 8 ]t11@int32 constC[1 1]@C[2 1]@t20@{R{Q1{C{Scint16}8}}}t10@{Q1{Bi32}}
      FunctionDecl=|
      | namespace SingleStream {
      | template < int NSamples, int ShiftAcc > 
      | void FIR_MultiKernel_cin::
      | filter(input_stream_cint16 * sin, input_stream< cacc48_t > * cin, output_stream_cint16 * sout);
      | }
      ClassDeclTypeOptions=|
      | C[1 1]@t93@namespace SingleStream {
      | template < int NSamples, int ShiftAcc > class FIR_MultiKernel_cin;
      | }
      ClassDecl=|
      | namespace SingleStream {
      | template < int NSamples, int ShiftAcc > class FIR_MultiKernel_cin;
      | }
  AIE Class Kernel18 : ModelComposer/AIE Class Kernel  KernelAllAttrs=|  PortNames={'sin'; 'cin'; 'sout'}  PortSerializedTypes={'{P{Tinput_stream{1{t{Scint16}}}}}'; '{P{Tinput_stream{1{t{Scacc48_t}}}}}'; '{P{Toutput_stream{1{t{Scint16}}}}}'}  PortWindowSizes={0.000000000000000000e+00; 0.000000000000000000e+00; 0.000000000000000000e+00}  PortWindowMargins={0.000000000000000000e+00; 0.000000000000000000e+00; 0.000000000000000000e+00}  PortSynchronicities={'auto'; 'auto'; 'auto'}  PortSignalSizes={0.000000000000000000e+00; 0.000000000000000000e+00; 4.000000000000000000e+00}  ClassTemplateSpecKind=implicit  ClassTemplateParamNames={'NSamples'; 'ShiftAcc'}  ClassTemplateParamKinds={'nontype'; 'nontype'}  ClassTemplateParamTypes={'int'; 'int'}  ClassTemplateParamValues={'512', '15'}  ClassCtorParamNames={'taps'; 'Delay'}  ClassCtorParamSerializedTypes={'{R{Q1{C{Scint16}8}}}'; '{Q1{Bi32}}'}  ClassCtorParamValues={'[14-121i 342-439i 1454-497i 8773+2748i 237+96i 102+525i -121+233i -54+21i]', '0'}  ClassIndex=1  ClassCtorIndex=1  ClassTabVisible=on  ClassTemplateParamsVisible=on  ClassCtorDeclVisible=on  ClassCtorParamsVisible=on  FunctionTabVisible=on  FunctionDecl=|  PortAttrs={ 'input', 'sin', 'input_stream_cint16 *', '', '', '', ''; 'input', 'cin', 'input_stream< cacc48_t > *', '', '', '', ''; 'output', 'sout', 'output_stream_cint16 *', '', '', '', 'N' }  PortAttrsEnables={'off', 'off', 'off', 'off', 'off', 'off', 'off';'off', 'off', 'off', 'off', 'off', 'off', 'off';'off', 'off', 'off', 'off', 'off', 'off', 'on'}  SampleTime=-1  ClassDeclTypeOptions=|  ClassDecl=|  ClassTemplateParams={ 'NSamples', 'int', 'BURST_LENGTH'; 'ShiftAcc', 'int', 'SHIFT_ACC' }  ClassTemplateParamsEnables={'off', 'off', 'on';'off', 'off', 'on'}  ClassCtorDeclTypeOptions=C[1 1]@t69@FIR_MultiKernel_cin(cint16 const ( & taps ) [ 8 ], int32 const Delay)  ClassCtorDecl=FIR_MultiKernel_cin(cint16 const ( & taps ) [ 8 ], int32 const Delay)  ClassCtorParams={ 'taps', 'cint16 const ( &) [ 8 ]', 'phi_3'; 'Delay', 'int32 const', '0' }  KernelHeaderFile=FirSingleStream.h  KernelClassName=SingleStream::FIR_MultiKernel_cin  KernelFunction=filter  KernelSourceFile=FirSingleStream.cpp  KernelSearchPaths={'$SRC', '$SRC/aie_kernels'}  PreProcOptions={}  CoreRuntimeRatio=0.9  KernelLocSpec=off  ColRowLocation=[25 0]  blockJsonConstraints="{\"type\":\"constraint\",\"constraintType\":\"coreUtilization\",\"sid\":\"385\",\"lhs\":{\"type\":\"runtimeRatio\",\"args\":{\"type\":\"kernel\",\"name\":\"SingleStreamSSR/SSR4/AIE Class Kernel18\",\"sid\":\"385\"}},\"rhs\":{\"type\":\"evaluable\",\"expr\":\"0.9\",\"value\":0.9},\"equality\":true}"  deprecateConstraints=1
      KernelAllAttrs=|
      | s[12;12;9;9;19;14;21;23;24;21;12;24;26;26;26;27;28;9;21;23;23;23;24;25;14;19;19;29]@FunctionNameDeclFileNamePortNamesPortTypesPortSerializedTypesPortDirectionsPortWindowSizeEnablesPortWindowMarginEnablesPortSynchronicityEnablesPortSignalSizeEnablesFunctionDeclFunctionTemplateSpecKindFunctionTemplateParamNamesFunctionTemplateParamKindsFunctionTemplateParamTypesFunctionTemplateParamValuesFunctionTemplateParamEnablesClassDeclClassTemplateSpecKindClassTemplateParamNamesClassTemplateParamKindsClassTemplateParamTypesClassTemplateParamValuesClassTemplateParamEnablesClassCtorDeclsClassCtorParamNamesClassCtorParamTypesClassCtorParamSerializedTypes[1 1]@C[28 1]@t6@filtert42@../../../src/aie_kernels/FirSingleStream.hC[3 1]@t3@sint3@cint4@soutC[3 1]@t21@input_stream_cint16 *t26@input_stream< cacc48_t > *t22@output_stream_cint16 *C[3 1]@t33@{P{Tinput_stream{1{t{Scint16}}}}}t35@{P{Tinput_stream{1{t{Scacc48_t}}}}}t34@{P{Toutput_stream{1{t{Scint16}}}}}C[3 1]@t5@inputt5@inputt6@outputC[3 1]@l0@l0@l0@C[3 1]@l0@l0@l0@C[3 1]@l0@l0@l0@C[3 1]@l0@l0@l1@t190@namespace SingleStream {
      | template < int NSamples, int ShiftAcc > 
      | void FIR_MultiKernel_cin::
      | filter(input_stream_cint16 * sin, input_stream< cacc48_t > * cin, output_stream_cint16 * sout);
      | }t4@nonee[0 1]@e[0 1]@e[0 1]@e[0 1]@e[0 1]@t93@namespace SingleStream {
      | template < int NSamples, int ShiftAcc > class FIR_MultiKernel_cin;
      | }t8@implicitC[2 1]@t8@NSamplest8@ShiftAccC[2 1]@t7@nontypet7@nontypeC[2 1]@t3@intt3@intC[2 1]@nnC[2 1]@l1@l1@C[1 1]@t69@FIR_MultiKernel_cin(cint16 const ( & taps ) [ 8 ], int32 const Delay)C[1 1]@C[2 1]@t4@tapst5@DelayC[1 1]@C[2 1]@t23@cint16 const ( &) [ 8 ]t11@int32 constC[1 1]@C[2 1]@t20@{R{Q1{C{Scint16}8}}}t10@{Q1{Bi32}}
      FunctionDecl=|
      | namespace SingleStream {
      | template < int NSamples, int ShiftAcc > 
      | void FIR_MultiKernel_cin::
      | filter(input_stream_cint16 * sin, input_stream< cacc48_t > * cin, output_stream_cint16 * sout);
      | }
      ClassDeclTypeOptions=|
      | C[1 1]@t93@namespace SingleStream {
      | template < int NSamples, int ShiftAcc > class FIR_MultiKernel_cin;
      | }
      ClassDecl=|
      | namespace SingleStream {
      | template < int NSamples, int ShiftAcc > class FIR_MultiKernel_cin;
      | }
  AIE Class Kernel3 : ModelComposer/AIE Class Kernel  KernelAllAttrs=|  PortNames={'sin'; 'cin'; 'cout'}  PortSerializedTypes={'{P{Tinput_stream{1{t{Scint16}}}}}'; '{P{Tinput_stream{1{t{Scacc48_t}}}}}'; '{P{Toutput_stream{1{t{Scacc48_t}}}}}'}  PortWindowSizes={0.000000000000000000e+00; 0.000000000000000000e+00; 0.000000000000000000e+00}  PortWindowMargins={0.000000000000000000e+00; 0.000000000000000000e+00; 0.000000000000000000e+00}  PortSynchronicities={'auto'; 'auto'; 'auto'}  PortSignalSizes={0.000000000000000000e+00; 0.000000000000000000e+00; 4.000000000000000000e+00}  ClassTemplateSpecKind=implicit  ClassTemplateParamNames={'NSamples'; 'ShiftAcc'}  ClassTemplateParamKinds={'nontype'; 'nontype'}  ClassTemplateParamTypes={'int'; 'int'}  ClassTemplateParamValues={'512', '15'}  ClassCtorParamNames={'taps'; 'Delay'}  ClassCtorParamSerializedTypes={'{R{Q1{C{Scint16}8}}}'; '{Q1{Bi32}}'}  ClassCtorParamValues={'[-21+26i 146-91i 1183+239i 4086+5221i 248-2878i 237-54i -160+111i -83-21i]', '0'}  ClassIndex=1  ClassCtorIndex=1  ClassTabVisible=on  ClassTemplateParamsVisible=on  ClassCtorDeclVisible=on  ClassCtorParamsVisible=on  FunctionTabVisible=on  FunctionDecl=|  PortAttrs={ 'input', 'sin', 'input_stream_cint16 *', '', '', '', ''; 'input', 'cin', 'input_stream< cacc48_t > *', '', '', '', ''; 'output', 'cout', 'output_stream< cacc48_t > *', '', '', '', 'N' }  PortAttrsEnables={'off', 'off', 'off', 'off', 'off', 'off', 'off';'off', 'off', 'off', 'off', 'off', 'off', 'off';'off', 'off', 'off', 'off', 'off', 'off', 'on'}  SampleTime=-1  ClassDeclTypeOptions=|  ClassDecl=|  ClassTemplateParams={ 'NSamples', 'int', 'BURST_LENGTH'; 'ShiftAcc', 'int', 'SHIFT_ACC' }  ClassTemplateParamsEnables={'off', 'off', 'on';'off', 'off', 'on'}  ClassCtorDeclTypeOptions=C[1 1]@t73@FIR_MultiKernel_cincout(cint16 const ( & taps ) [ 8 ], int32 const Delay)  ClassCtorDecl=FIR_MultiKernel_cincout(cint16 const ( & taps ) [ 8 ], int32 const Delay)  ClassCtorParams={ 'taps', 'cint16 const ( &) [ 8 ]', 'phi_2'; 'Delay', 'int32 const', '0' }  KernelHeaderFile=FirSingleStream.h  KernelClassName=SingleStream::FIR_MultiKernel_cincout  KernelFunction=filter  KernelSourceFile=FirSingleStream.cpp  KernelSearchPaths={'$SRC', '$SRC/aie_kernels'}  PreProcOptions={}  CoreRuntimeRatio=0.9  KernelLocSpec=off  ColRowLocation=[25 0]  blockJsonConstraints="{\"type\":\"constraint\",\"constraintType\":\"coreUtilization\",\"sid\":\"398\",\"lhs\":{\"type\":\"runtimeRatio\",\"args\":{\"type\":\"kernel\",\"name\":\"SingleStreamSSR/SSR4/AIE Class Kernel3\",\"sid\":\"398\"}},\"rhs\":{\"type\":\"evaluable\",\"expr\":\"0.9\",\"value\":0.9},\"equality\":true}"  deprecateConstraints=1
      KernelAllAttrs=|
      | s[12;12;9;9;19;14;21;23;24;21;12;24;26;26;26;27;28;9;21;23;23;23;24;25;14;19;19;29]@FunctionNameDeclFileNamePortNamesPortTypesPortSerializedTypesPortDirectionsPortWindowSizeEnablesPortWindowMarginEnablesPortSynchronicityEnablesPortSignalSizeEnablesFunctionDeclFunctionTemplateSpecKindFunctionTemplateParamNamesFunctionTemplateParamKindsFunctionTemplateParamTypesFunctionTemplateParamValuesFunctionTemplateParamEnablesClassDeclClassTemplateSpecKindClassTemplateParamNamesClassTemplateParamKindsClassTemplateParamTypesClassTemplateParamValuesClassTemplateParamEnablesClassCtorDeclsClassCtorParamNamesClassCtorParamTypesClassCtorParamSerializedTypes[1 1]@C[28 1]@t6@filtert42@../../../src/aie_kernels/FirSingleStream.hC[3 1]@t3@sint3@cint4@coutC[3 1]@t21@input_stream_cint16 *t26@input_stream< cacc48_t > *t27@output_stream< cacc48_t > *C[3 1]@t33@{P{Tinput_stream{1{t{Scint16}}}}}t35@{P{Tinput_stream{1{t{Scacc48_t}}}}}t36@{P{Toutput_stream{1{t{Scacc48_t}}}}}C[3 1]@t5@inputt5@inputt6@outputC[3 1]@l0@l0@l0@C[3 1]@l0@l0@l0@C[3 1]@l0@l0@l0@C[3 1]@l0@l0@l1@t199@namespace SingleStream {
      | template < int NSamples, int ShiftAcc > 
      | void FIR_MultiKernel_cincout::
      | filter(input_stream_cint16 * sin, input_stream< cacc48_t > * cin, output_stream< cacc48_t > * cout);
      | }t4@nonee[0 1]@e[0 1]@e[0 1]@e[0 1]@e[0 1]@t97@namespace SingleStream {
      | template < int NSamples, int ShiftAcc > class FIR_MultiKernel_cincout;
      | }t8@implicitC[2 1]@t8@NSamplest8@ShiftAccC[2 1]@t7@nontypet7@nontypeC[2 1]@t3@intt3@intC[2 1]@nnC[2 1]@l1@l1@C[1 1]@t73@FIR_MultiKernel_cincout(cint16 const ( & taps ) [ 8 ], int32 const Delay)C[1 1]@C[2 1]@t4@tapst5@DelayC[1 1]@C[2 1]@t23@cint16 const ( &) [ 8 ]t11@int32 constC[1 1]@C[2 1]@t20@{R{Q1{C{Scint16}8}}}t10@{Q1{Bi32}}
      FunctionDecl=|
      | namespace SingleStream {
      | template < int NSamples, int ShiftAcc > 
      | void FIR_MultiKernel_cincout::
      | filter(input_stream_cint16 * sin, input_stream< cacc48_t > * cin, output_stream< cacc48_t > * cout);
      | }
      ClassDeclTypeOptions=|
      | C[1 1]@t97@namespace SingleStream {
      | template < int NSamples, int ShiftAcc > class FIR_MultiKernel_cincout;
      | }
      ClassDecl=|
      | namespace SingleStream {
      | template < int NSamples, int ShiftAcc > class FIR_MultiKernel_cincout;
      | }
  AIE Class Kernel4 : ModelComposer/AIE Class Kernel  KernelAllAttrs=|  PortNames={'sin'; 'cout'}  PortSerializedTypes={'{P{Tinput_stream{1{t{Scint16}}}}}'; '{P{Toutput_stream{1{t{Scacc48_t}}}}}'}  PortWindowSizes={0.000000000000000000e+00; 0.000000000000000000e+00}  PortWindowMargins={0.000000000000000000e+00; 0.000000000000000000e+00}  PortSynchronicities={'auto'; 'auto'}  PortSignalSizes={0.000000000000000000e+00; 4.000000000000000000e+00}  ClassTemplateSpecKind=implicit  ClassTemplateParamNames={'NSamples'; 'ShiftAcc'}  ClassTemplateParamKinds={'nontype'; 'nontype'}  ClassTemplateParamTypes={'int'; 'int'}  ClassTemplateParamValues={'512', '15'}  ClassCtorParamNames={'taps'; 'Delay'}  ClassCtorParamSerializedTypes={'{R{Q1{C{Scint16}8}}}'; '{Q1{Bi32}}'}  ClassCtorParamValues={'[-54-21i -121-233i 102-525i 237-96i 8773-2748i 1454+497i 342+439i 14+121i]', '0'}  ClassIndex=1  ClassCtorIndex=1  ClassTabVisible=on  ClassTemplateParamsVisible=on  ClassCtorDeclVisible=on  ClassCtorParamsVisible=on  FunctionTabVisible=on  FunctionDecl=|  PortAttrs={ 'input', 'sin', 'input_stream_cint16 *', '', '', '', ''; 'output', 'cout', 'output_stream< cacc48_t > *', '', '', '', 'N' }  PortAttrsEnables={'off', 'off', 'off', 'off', 'off', 'off', 'off';'off', 'off', 'off', 'off', 'off', 'off', 'on'}  SampleTime=-1  ClassDeclTypeOptions=|  ClassDecl=|  ClassTemplateParams={ 'NSamples', 'int', 'BURST_LENGTH'; 'ShiftAcc', 'int', 'SHIFT_ACC' }  ClassTemplateParamsEnables={'off', 'off', 'on';'off', 'off', 'on'}  ClassCtorDeclTypeOptions=C[1 1]@t70@FIR_MultiKernel_cout(cint16 const ( & taps ) [ 8 ], int32 const Delay)  ClassCtorDecl=FIR_MultiKernel_cout(cint16 const ( & taps ) [ 8 ], int32 const Delay)  ClassCtorParams={ 'taps', 'cint16 const ( &) [ 8 ]', 'phi_0'; 'Delay', 'int32 const', '0' }  KernelHeaderFile=FirSingleStream.h  KernelClassName=SingleStream::FIR_MultiKernel_cout  KernelFunction=filter  KernelSourceFile=FirSingleStream.cpp  KernelSearchPaths={'$SRC', '$SRC/aie_kernels'}  PreProcOptions={}  CoreRuntimeRatio=0.9  KernelLocSpec=on  ColRowLocation=LOCATION_2_0  blockJsonConstraints="[{\"type\":\"constraint\",\"constraintType\":\"coreUtilization\",\"sid\":\"387\",\"lhs\":{\"type\":\"runtimeRatio\",\"args\":{\"type\":\"kernel\",\"name\":\"SingleStreamSSR/SSR4/AIE Class Kernel4\",\"sid\":\"387\"}},\"rhs\":{\"type\":\"evaluable\",\"expr\":\"0.9\",\"value\":0.9},\"equality\":true},{\"type\":\"constraint\",\"constraintType\":\"location_kernel\",\"sid\":\"387\",\"lhs\":{\"type\":\"location\",\"templParam\":\"kernel\",\"args\":{\"type\":\"kernel\",\"name\":\"SingleStreamSSR/SSR4/AIE Class Kernel4\",\"sid\":\"387\"}},\"rhs\":{\"type\":\"tile\",\"args\":[{\"type\":\"evaluable\",\"expr\":\"28\",\"value\":28},{\"type\":\"evaluable\",\"expr\":\"3\",\"value\":3}]},\"equality\":true}]"  deprecateConstraints=1
      KernelAllAttrs=|
      | s[12;12;9;9;19;14;21;23;24;21;12;24;26;26;26;27;28;9;21;23;23;23;24;25;14;19;19;29]@FunctionNameDeclFileNamePortNamesPortTypesPortSerializedTypesPortDirectionsPortWindowSizeEnablesPortWindowMarginEnablesPortSynchronicityEnablesPortSignalSizeEnablesFunctionDeclFunctionTemplateSpecKindFunctionTemplateParamNamesFunctionTemplateParamKindsFunctionTemplateParamTypesFunctionTemplateParamValuesFunctionTemplateParamEnablesClassDeclClassTemplateSpecKindClassTemplateParamNamesClassTemplateParamKindsClassTemplateParamTypesClassTemplateParamValuesClassTemplateParamEnablesClassCtorDeclsClassCtorParamNamesClassCtorParamTypesClassCtorParamSerializedTypes[1 1]@C[28 1]@t6@filtert42@../../../src/aie_kernels/FirSingleStream.hC[2 1]@t3@sint4@coutC[2 1]@t21@input_stream_cint16 *t27@output_stream< cacc48_t > *C[2 1]@t33@{P{Tinput_stream{1{t{Scint16}}}}}t36@{P{Toutput_stream{1{t{Scacc48_t}}}}}C[2 1]@t5@inputt6@outputC[2 1]@l0@l0@C[2 1]@l0@l0@C[2 1]@l0@l0@C[2 1]@l0@l1@t164@namespace SingleStream {
      | template < int NSamples, int ShiftAcc > 
      | void FIR_MultiKernel_cout::
      | filter(input_stream_cint16 * sin, output_stream< cacc48_t > * cout);
      | }t4@nonee[0 1]@e[0 1]@e[0 1]@e[0 1]@e[0 1]@t94@namespace SingleStream {
      | template < int NSamples, int ShiftAcc > class FIR_MultiKernel_cout;
      | }t8@implicitC[2 1]@t8@NSamplest8@ShiftAccC[2 1]@t7@nontypet7@nontypeC[2 1]@t3@intt3@intC[2 1]@nnC[2 1]@l1@l1@C[1 1]@t70@FIR_MultiKernel_cout(cint16 const ( & taps ) [ 8 ], int32 const Delay)C[1 1]@C[2 1]@t4@tapst5@DelayC[1 1]@C[2 1]@t23@cint16 const ( &) [ 8 ]t11@int32 constC[1 1]@C[2 1]@t20@{R{Q1{C{Scint16}8}}}t10@{Q1{Bi32}}
      FunctionDecl=|
      | namespace SingleStream {
      | template < int NSamples, int ShiftAcc > 
      | void FIR_MultiKernel_cout::
      | filter(input_stream_cint16 * sin, output_stream< cacc48_t > * cout);
      | }
      ClassDeclTypeOptions=|
      | C[1 1]@t94@namespace SingleStream {
      | template < int NSamples, int ShiftAcc > class FIR_MultiKernel_cout;
      | }
      ClassDecl=|
      | namespace SingleStream {
      | template < int NSamples, int ShiftAcc > class FIR_MultiKernel_cout;
      | }
  AIE Class Kernel5 : ModelComposer/AIE Class Kernel  KernelAllAttrs=|  PortNames={'sin'; 'cin'; 'cout'}  PortSerializedTypes={'{P{Tinput_stream{1{t{Scint16}}}}}'; '{P{Tinput_stream{1{t{Scacc48_t}}}}}'; '{P{Toutput_stream{1{t{Scacc48_t}}}}}'}  PortWindowSizes={0.000000000000000000e+00; 0.000000000000000000e+00; 0.000000000000000000e+00}  PortWindowMargins={0.000000000000000000e+00; 0.000000000000000000e+00; 0.000000000000000000e+00}  PortSynchronicities={'auto'; 'auto'; 'auto'}  PortSignalSizes={0.000000000000000000e+00; 0.000000000000000000e+00; 4.000000000000000000e+00}  ClassTemplateSpecKind=implicit  ClassTemplateParamNames={'NSamples'; 'ShiftAcc'}  ClassTemplateParamKinds={'nontype'; 'nontype'}  ClassTemplateParamTypes={'int'; 'int'}  ClassTemplateParamValues={'512', '15'}  ClassCtorParamNames={'taps'; 'Delay'}  ClassCtorParamSerializedTypes={'{R{Q1{C{Scint16}8}}}'; '{Q1{Bi32}}'}  ClassCtorParamValues={'[-83+21i -160-111i 237+54i 248+2878i 4086-5221i 1183-239i 146+91i -21-26i]', '0'}  ClassIndex=1  ClassCtorIndex=1  ClassTabVisible=on  ClassTemplateParamsVisible=on  ClassCtorDeclVisible=on  ClassCtorParamsVisible=on  FunctionTabVisible=on  FunctionDecl=|  PortAttrs={ 'input', 'sin', 'input_stream_cint16 *', '', '', '', ''; 'input', 'cin', 'input_stream< cacc48_t > *', '', '', '', ''; 'output', 'cout', 'output_stream< cacc48_t > *', '', '', '', 'N' }  PortAttrsEnables={'off', 'off', 'off', 'off', 'off', 'off', 'off';'off', 'off', 'off', 'off', 'off', 'off', 'off';'off', 'off', 'off', 'off', 'off', 'off', 'on'}  SampleTime=-1  ClassDeclTypeOptions=|  ClassDecl=|  ClassTemplateParams={ 'NSamples', 'int', 'BURST_LENGTH'; 'ShiftAcc', 'int', 'SHIFT_ACC' }  ClassTemplateParamsEnables={'off', 'off', 'on';'off', 'off', 'on'}  ClassCtorDeclTypeOptions=C[1 1]@t73@FIR_MultiKernel_cincout(cint16 const ( & taps ) [ 8 ], int32 const Delay)  ClassCtorDecl=FIR_MultiKernel_cincout(cint16 const ( & taps ) [ 8 ], int32 const Delay)  ClassCtorParams={ 'taps', 'cint16 const ( &) [ 8 ]', 'phi_1'; 'Delay', 'int32 const', '0' }  KernelHeaderFile=FirSingleStream.h  KernelClassName=SingleStream::FIR_MultiKernel_cincout  KernelFunction=filter  KernelSourceFile=FirSingleStream.cpp  KernelSearchPaths={'$SRC', '$SRC/aie_kernels'}  PreProcOptions={}  CoreRuntimeRatio=0.9  KernelLocSpec=off  ColRowLocation=[25 0]  blockJsonConstraints="{\"type\":\"constraint\",\"constraintType\":\"coreUtilization\",\"sid\":\"394\",\"lhs\":{\"type\":\"runtimeRatio\",\"args\":{\"type\":\"kernel\",\"name\":\"SingleStreamSSR/SSR4/AIE Class Kernel5\",\"sid\":\"394\"}},\"rhs\":{\"type\":\"evaluable\",\"expr\":\"0.9\",\"value\":0.9},\"equality\":true}"  deprecateConstraints=1
      KernelAllAttrs=|
      | s[12;12;9;9;19;14;21;23;24;21;12;24;26;26;26;27;28;9;21;23;23;23;24;25;14;19;19;29]@FunctionNameDeclFileNamePortNamesPortTypesPortSerializedTypesPortDirectionsPortWindowSizeEnablesPortWindowMarginEnablesPortSynchronicityEnablesPortSignalSizeEnablesFunctionDeclFunctionTemplateSpecKindFunctionTemplateParamNamesFunctionTemplateParamKindsFunctionTemplateParamTypesFunctionTemplateParamValuesFunctionTemplateParamEnablesClassDeclClassTemplateSpecKindClassTemplateParamNamesClassTemplateParamKindsClassTemplateParamTypesClassTemplateParamValuesClassTemplateParamEnablesClassCtorDeclsClassCtorParamNamesClassCtorParamTypesClassCtorParamSerializedTypes[1 1]@C[28 1]@t6@filtert42@../../../src/aie_kernels/FirSingleStream.hC[3 1]@t3@sint3@cint4@coutC[3 1]@t21@input_stream_cint16 *t26@input_stream< cacc48_t > *t27@output_stream< cacc48_t > *C[3 1]@t33@{P{Tinput_stream{1{t{Scint16}}}}}t35@{P{Tinput_stream{1{t{Scacc48_t}}}}}t36@{P{Toutput_stream{1{t{Scacc48_t}}}}}C[3 1]@t5@inputt5@inputt6@outputC[3 1]@l0@l0@l0@C[3 1]@l0@l0@l0@C[3 1]@l0@l0@l0@C[3 1]@l0@l0@l1@t199@namespace SingleStream {
      | template < int NSamples, int ShiftAcc > 
      | void FIR_MultiKernel_cincout::
      | filter(input_stream_cint16 * sin, input_stream< cacc48_t > * cin, output_stream< cacc48_t > * cout);
      | }t4@nonee[0 1]@e[0 1]@e[0 1]@e[0 1]@e[0 1]@t97@namespace SingleStream {
      | template < int NSamples, int ShiftAcc > class FIR_MultiKernel_cincout;
      | }t8@implicitC[2 1]@t8@NSamplest8@ShiftAccC[2 1]@t7@nontypet7@nontypeC[2 1]@t3@intt3@intC[2 1]@nnC[2 1]@l1@l1@C[1 1]@t73@FIR_MultiKernel_cincout(cint16 const ( & taps ) [ 8 ], int32 const Delay)C[1 1]@C[2 1]@t4@tapst5@DelayC[1 1]@C[2 1]@t23@cint16 const ( &) [ 8 ]t11@int32 constC[1 1]@C[2 1]@t20@{R{Q1{C{Scint16}8}}}t10@{Q1{Bi32}}
      FunctionDecl=|
      | namespace SingleStream {
      | template < int NSamples, int ShiftAcc > 
      | void FIR_MultiKernel_cincout::
      | filter(input_stream_cint16 * sin, input_stream< cacc48_t > * cin, output_stream< cacc48_t > * cout);
      | }
      ClassDeclTypeOptions=|
      | C[1 1]@t97@namespace SingleStream {
      | template < int NSamples, int ShiftAcc > class FIR_MultiKernel_cincout;
      | }
      ClassDecl=|
      | namespace SingleStream {
      | template < int NSamples, int ShiftAcc > class FIR_MultiKernel_cincout;
      | }
  AIE Class Kernel6 : ModelComposer/AIE Class Kernel  KernelAllAttrs=|  PortNames={'sin'; 'cin'; 'cout'}  PortSerializedTypes={'{P{Tinput_stream{1{t{Scint16}}}}}'; '{P{Tinput_stream{1{t{Scacc48_t}}}}}'; '{P{Toutput_stream{1{t{Scacc48_t}}}}}'}  PortWindowSizes={0.000000000000000000e+00; 0.000000000000000000e+00; 0.000000000000000000e+00}  PortWindowMargins={0.000000000000000000e+00; 0.000000000000000000e+00; 0.000000000000000000e+00}  PortSynchronicities={'auto'; 'auto'; 'auto'}  PortSignalSizes={0.000000000000000000e+00; 0.000000000000000000e+00; 4.000000000000000000e+00}  ClassTemplateSpecKind=implicit  ClassTemplateParamNames={'NSamples'; 'ShiftAcc'}  ClassTemplateParamKinds={'nontype'; 'nontype'}  ClassTemplateParamTypes={'int'; 'int'}  ClassTemplateParamValues={'512', '15'}  ClassCtorParamNames={'taps'; 'Delay'}  ClassCtorParamSerializedTypes={'{R{Q1{C{Scint16}8}}}'; '{Q1{Bi32}}'}  ClassCtorParamValues={'[14-121i 342-439i 1454-497i 8773+2748i 237+96i 102+525i -121+233i -54+21i]', '1'}  ClassIndex=1  ClassCtorIndex=1  ClassTabVisible=on  ClassTemplateParamsVisible=on  ClassCtorDeclVisible=on  ClassCtorParamsVisible=on  FunctionTabVisible=on  FunctionDecl=|  PortAttrs={ 'input', 'sin', 'input_stream_cint16 *', '', '', '', ''; 'input', 'cin', 'input_stream< cacc48_t > *', '', '', '', ''; 'output', 'cout', 'output_stream< cacc48_t > *', '', '', '', 'N' }  PortAttrsEnables={'off', 'off', 'off', 'off', 'off', 'off', 'off';'off', 'off', 'off', 'off', 'off', 'off', 'off';'off', 'off', 'off', 'off', 'off', 'off', 'on'}  SampleTime=-1  ClassDeclTypeOptions=|  ClassDecl=|  ClassTemplateParams={ 'NSamples', 'int', 'BURST_LENGTH'; 'ShiftAcc', 'int', 'SHIFT_ACC' }  ClassTemplateParamsEnables={'off', 'off', 'on';'off', 'off', 'on'}  ClassCtorDeclTypeOptions=C[1 1]@t73@FIR_MultiKernel_cincout(cint16 const ( & taps ) [ 8 ], int32 const Delay)  ClassCtorDecl=FIR_MultiKernel_cincout(cint16 const ( & taps ) [ 8 ], int32 const Delay)  ClassCtorParams={ 'taps', 'cint16 const ( &) [ 8 ]', 'phi_3'; 'Delay', 'int32 const', '1' }  KernelHeaderFile=FirSingleStream.h  KernelClassName=SingleStream::FIR_MultiKernel_cincout  KernelFunction=filter  KernelSourceFile=FirSingleStream.cpp  KernelSearchPaths={'$SRC', '$SRC/aie_kernels'}  PreProcOptions={}  CoreRuntimeRatio=0.9  KernelLocSpec=off  ColRowLocation=[25 0]  blockJsonConstraints="{\"type\":\"constraint\",\"constraintType\":\"coreUtilization\",\"sid\":\"395\",\"lhs\":{\"type\":\"runtimeRatio\",\"args\":{\"type\":\"kernel\",\"name\":\"SingleStreamSSR/SSR4/AIE Class Kernel6\",\"sid\":\"395\"}},\"rhs\":{\"type\":\"evaluable\",\"expr\":\"0.9\",\"value\":0.9},\"equality\":true}"  deprecateConstraints=1
      KernelAllAttrs=|
      | s[12;12;9;9;19;14;21;23;24;21;12;24;26;26;26;27;28;9;21;23;23;23;24;25;14;19;19;29]@FunctionNameDeclFileNamePortNamesPortTypesPortSerializedTypesPortDirectionsPortWindowSizeEnablesPortWindowMarginEnablesPortSynchronicityEnablesPortSignalSizeEnablesFunctionDeclFunctionTemplateSpecKindFunctionTemplateParamNamesFunctionTemplateParamKindsFunctionTemplateParamTypesFunctionTemplateParamValuesFunctionTemplateParamEnablesClassDeclClassTemplateSpecKindClassTemplateParamNamesClassTemplateParamKindsClassTemplateParamTypesClassTemplateParamValuesClassTemplateParamEnablesClassCtorDeclsClassCtorParamNamesClassCtorParamTypesClassCtorParamSerializedTypes[1 1]@C[28 1]@t6@filtert42@../../../src/aie_kernels/FirSingleStream.hC[3 1]@t3@sint3@cint4@coutC[3 1]@t21@input_stream_cint16 *t26@input_stream< cacc48_t > *t27@output_stream< cacc48_t > *C[3 1]@t33@{P{Tinput_stream{1{t{Scint16}}}}}t35@{P{Tinput_stream{1{t{Scacc48_t}}}}}t36@{P{Toutput_stream{1{t{Scacc48_t}}}}}C[3 1]@t5@inputt5@inputt6@outputC[3 1]@l0@l0@l0@C[3 1]@l0@l0@l0@C[3 1]@l0@l0@l0@C[3 1]@l0@l0@l1@t199@namespace SingleStream {
      | template < int NSamples, int ShiftAcc > 
      | void FIR_MultiKernel_cincout::
      | filter(input_stream_cint16 * sin, input_stream< cacc48_t > * cin, output_stream< cacc48_t > * cout);
      | }t4@nonee[0 1]@e[0 1]@e[0 1]@e[0 1]@e[0 1]@t97@namespace SingleStream {
      | template < int NSamples, int ShiftAcc > class FIR_MultiKernel_cincout;
      | }t8@implicitC[2 1]@t8@NSamplest8@ShiftAccC[2 1]@t7@nontypet7@nontypeC[2 1]@t3@intt3@intC[2 1]@nnC[2 1]@l1@l1@C[1 1]@t73@FIR_MultiKernel_cincout(cint16 const ( & taps ) [ 8 ], int32 const Delay)C[1 1]@C[2 1]@t4@tapst5@DelayC[1 1]@C[2 1]@t23@cint16 const ( &) [ 8 ]t11@int32 constC[1 1]@C[2 1]@t20@{R{Q1{C{Scint16}8}}}t10@{Q1{Bi32}}
      FunctionDecl=|
      | namespace SingleStream {
      | template < int NSamples, int ShiftAcc > 
      | void FIR_MultiKernel_cincout::
      | filter(input_stream_cint16 * sin, input_stream< cacc48_t > * cin, output_stream< cacc48_t > * cout);
      | }
      ClassDeclTypeOptions=|
      | C[1 1]@t97@namespace SingleStream {
      | template < int NSamples, int ShiftAcc > class FIR_MultiKernel_cincout;
      | }
      ClassDecl=|
      | namespace SingleStream {
      | template < int NSamples, int ShiftAcc > class FIR_MultiKernel_cincout;
      | }
  AIE Class Kernel7 : ModelComposer/AIE Class Kernel  KernelAllAttrs=|  PortNames={'sin'; 'cin'; 'cout'}  PortSerializedTypes={'{P{Tinput_stream{1{t{Scint16}}}}}'; '{P{Tinput_stream{1{t{Scacc48_t}}}}}'; '{P{Toutput_stream{1{t{Scacc48_t}}}}}'}  PortWindowSizes={0.000000000000000000e+00; 0.000000000000000000e+00; 0.000000000000000000e+00}  PortWindowMargins={0.000000000000000000e+00; 0.000000000000000000e+00; 0.000000000000000000e+00}  PortSynchronicities={'auto'; 'auto'; 'auto'}  PortSignalSizes={0.000000000000000000e+00; 0.000000000000000000e+00; 4.000000000000000000e+00}  ClassTemplateSpecKind=implicit  ClassTemplateParamNames={'NSamples'; 'ShiftAcc'}  ClassTemplateParamKinds={'nontype'; 'nontype'}  ClassTemplateParamTypes={'int'; 'int'}  ClassTemplateParamValues={'512', '15'}  ClassCtorParamNames={'taps'; 'Delay'}  ClassCtorParamSerializedTypes={'{R{Q1{C{Scint16}8}}}'; '{Q1{Bi32}}'}  ClassCtorParamValues={'[-54-21i -121-233i 102-525i 237-96i 8773-2748i 1454+497i 342+439i 14+121i]', '0'}  ClassIndex=1  ClassCtorIndex=1  ClassTabVisible=on  ClassTemplateParamsVisible=on  ClassCtorDeclVisible=on  ClassCtorParamsVisible=on  FunctionTabVisible=on  FunctionDecl=|  PortAttrs={ 'input', 'sin', 'input_stream_cint16 *', '', '', '', ''; 'input', 'cin', 'input_stream< cacc48_t > *', '', '', '', ''; 'output', 'cout', 'output_stream< cacc48_t > *', '', '', '', 'N' }  PortAttrsEnables={'off', 'off', 'off', 'off', 'off', 'off', 'off';'off', 'off', 'off', 'off', 'off', 'off', 'off';'off', 'off', 'off', 'off', 'off', 'off', 'on'}  SampleTime=-1  ClassDeclTypeOptions=|  ClassDecl=|  ClassTemplateParams={ 'NSamples', 'int', 'BURST_LENGTH'; 'ShiftAcc', 'int', 'SHIFT_ACC' }  ClassTemplateParamsEnables={'off', 'off', 'on';'off', 'off', 'on'}  ClassCtorDeclTypeOptions=C[1 1]@t73@FIR_MultiKernel_cincout(cint16 const ( & taps ) [ 8 ], int32 const Delay)  ClassCtorDecl=FIR_MultiKernel_cincout(cint16 const ( & taps ) [ 8 ], int32 const Delay)  ClassCtorParams={ 'taps', 'cint16 const ( &) [ 8 ]', 'phi_0'; 'Delay', 'int32 const', '0' }  KernelHeaderFile=FirSingleStream.h  KernelClassName=SingleStream::FIR_MultiKernel_cincout  KernelFunction=filter  KernelSourceFile=FirSingleStream.cpp  KernelSearchPaths={'$SRC', '$SRC/aie_kernels'}  PreProcOptions={}  CoreRuntimeRatio=0.9  KernelLocSpec=off  ColRowLocation=[25 0]  blockJsonConstraints="{\"type\":\"constraint\",\"constraintType\":\"coreUtilization\",\"sid\":\"397\",\"lhs\":{\"type\":\"runtimeRatio\",\"args\":{\"type\":\"kernel\",\"name\":\"SingleStreamSSR/SSR4/AIE Class Kernel7\",\"sid\":\"397\"}},\"rhs\":{\"type\":\"evaluable\",\"expr\":\"0.9\",\"value\":0.9},\"equality\":true}"  deprecateConstraints=1
      KernelAllAttrs=|
      | s[12;12;9;9;19;14;21;23;24;21;12;24;26;26;26;27;28;9;21;23;23;23;24;25;14;19;19;29]@FunctionNameDeclFileNamePortNamesPortTypesPortSerializedTypesPortDirectionsPortWindowSizeEnablesPortWindowMarginEnablesPortSynchronicityEnablesPortSignalSizeEnablesFunctionDeclFunctionTemplateSpecKindFunctionTemplateParamNamesFunctionTemplateParamKindsFunctionTemplateParamTypesFunctionTemplateParamValuesFunctionTemplateParamEnablesClassDeclClassTemplateSpecKindClassTemplateParamNamesClassTemplateParamKindsClassTemplateParamTypesClassTemplateParamValuesClassTemplateParamEnablesClassCtorDeclsClassCtorParamNamesClassCtorParamTypesClassCtorParamSerializedTypes[1 1]@C[28 1]@t6@filtert42@../../../src/aie_kernels/FirSingleStream.hC[3 1]@t3@sint3@cint4@coutC[3 1]@t21@input_stream_cint16 *t26@input_stream< cacc48_t > *t27@output_stream< cacc48_t > *C[3 1]@t33@{P{Tinput_stream{1{t{Scint16}}}}}t35@{P{Tinput_stream{1{t{Scacc48_t}}}}}t36@{P{Toutput_stream{1{t{Scacc48_t}}}}}C[3 1]@t5@inputt5@inputt6@outputC[3 1]@l0@l0@l0@C[3 1]@l0@l0@l0@C[3 1]@l0@l0@l0@C[3 1]@l0@l0@l1@t199@namespace SingleStream {
      | template < int NSamples, int ShiftAcc > 
      | void FIR_MultiKernel_cincout::
      | filter(input_stream_cint16 * sin, input_stream< cacc48_t > * cin, output_stream< cacc48_t > * cout);
      | }t4@nonee[0 1]@e[0 1]@e[0 1]@e[0 1]@e[0 1]@t97@namespace SingleStream {
      | template < int NSamples, int ShiftAcc > class FIR_MultiKernel_cincout;
      | }t8@implicitC[2 1]@t8@NSamplest8@ShiftAccC[2 1]@t7@nontypet7@nontypeC[2 1]@t3@intt3@intC[2 1]@nnC[2 1]@l1@l1@C[1 1]@t73@FIR_MultiKernel_cincout(cint16 const ( & taps ) [ 8 ], int32 const Delay)C[1 1]@C[2 1]@t4@tapst5@DelayC[1 1]@C[2 1]@t23@cint16 const ( &) [ 8 ]t11@int32 constC[1 1]@C[2 1]@t20@{R{Q1{C{Scint16}8}}}t10@{Q1{Bi32}}
      FunctionDecl=|
      | namespace SingleStream {
      | template < int NSamples, int ShiftAcc > 
      | void FIR_MultiKernel_cincout::
      | filter(input_stream_cint16 * sin, input_stream< cacc48_t > * cin, output_stream< cacc48_t > * cout);
      | }
      ClassDeclTypeOptions=|
      | C[1 1]@t97@namespace SingleStream {
      | template < int NSamples, int ShiftAcc > class FIR_MultiKernel_cincout;
      | }
      ClassDecl=|
      | namespace SingleStream {
      | template < int NSamples, int ShiftAcc > class FIR_MultiKernel_cincout;
      | }
  AIE Class Kernel8 : ModelComposer/AIE Class Kernel  KernelAllAttrs=|  PortNames={'sin'; 'cin'; 'sout'}  PortSerializedTypes={'{P{Tinput_stream{1{t{Scint16}}}}}'; '{P{Tinput_stream{1{t{Scacc48_t}}}}}'; '{P{Toutput_stream{1{t{Scint16}}}}}'}  PortWindowSizes={0.000000000000000000e+00; 0.000000000000000000e+00; 0.000000000000000000e+00}  PortWindowMargins={0.000000000000000000e+00; 0.000000000000000000e+00; 0.000000000000000000e+00}  PortSynchronicities={'auto'; 'auto'; 'auto'}  PortSignalSizes={0.000000000000000000e+00; 0.000000000000000000e+00; 4.000000000000000000e+00}  ClassTemplateSpecKind=implicit  ClassTemplateParamNames={'NSamples'; 'ShiftAcc'}  ClassTemplateParamKinds={'nontype'; 'nontype'}  ClassTemplateParamTypes={'int'; 'int'}  ClassTemplateParamValues={'512', '15'}  ClassCtorParamNames={'taps'; 'Delay'}  ClassCtorParamSerializedTypes={'{R{Q1{C{Scint16}8}}}'; '{Q1{Bi32}}'}  ClassCtorParamValues={'[-83+21i -160-111i 237+54i 248+2878i 4086-5221i 1183-239i 146+91i -21-26i]', '0'}  ClassIndex=1  ClassCtorIndex=1  ClassTabVisible=on  ClassTemplateParamsVisible=on  ClassCtorDeclVisible=on  ClassCtorParamsVisible=on  FunctionTabVisible=on  FunctionDecl=|  PortAttrs={ 'input', 'sin', 'input_stream_cint16 *', '', '', '', ''; 'input', 'cin', 'input_stream< cacc48_t > *', '', '', '', ''; 'output', 'sout', 'output_stream_cint16 *', '', '', '', 'N' }  PortAttrsEnables={'off', 'off', 'off', 'off', 'off', 'off', 'off';'off', 'off', 'off', 'off', 'off', 'off', 'off';'off', 'off', 'off', 'off', 'off', 'off', 'on'}  SampleTime=-1  ClassDeclTypeOptions=|  ClassDecl=|  ClassTemplateParams={ 'NSamples', 'int', 'BURST_LENGTH'; 'ShiftAcc', 'int', 'SHIFT_ACC' }  ClassTemplateParamsEnables={'off', 'off', 'on';'off', 'off', 'on'}  ClassCtorDeclTypeOptions=C[1 1]@t69@FIR_MultiKernel_cin(cint16 const ( & taps ) [ 8 ], int32 const Delay)  ClassCtorDecl=FIR_MultiKernel_cin(cint16 const ( & taps ) [ 8 ], int32 const Delay)  ClassCtorParams={ 'taps', 'cint16 const ( &) [ 8 ]', 'phi_1'; 'Delay', 'int32 const', '0' }  KernelHeaderFile=FirSingleStream.h  KernelClassName=SingleStream::FIR_MultiKernel_cin  KernelFunction=filter  KernelSourceFile=FirSingleStream.cpp  KernelSearchPaths={'$SRC', '$SRC/aie_kernels'}  PreProcOptions={}  CoreRuntimeRatio=0.9  KernelLocSpec=off  ColRowLocation=[25 0]  blockJsonConstraints="{\"type\":\"constraint\",\"constraintType\":\"coreUtilization\",\"sid\":\"384\",\"lhs\":{\"type\":\"runtimeRatio\",\"args\":{\"type\":\"kernel\",\"name\":\"SingleStreamSSR/SSR4/AIE Class Kernel8\",\"sid\":\"384\"}},\"rhs\":{\"type\":\"evaluable\",\"expr\":\"0.9\",\"value\":0.9},\"equality\":true}"  deprecateConstraints=1
      KernelAllAttrs=|
      | s[12;12;9;9;19;14;21;23;24;21;12;24;26;26;26;27;28;9;21;23;23;23;24;25;14;19;19;29]@FunctionNameDeclFileNamePortNamesPortTypesPortSerializedTypesPortDirectionsPortWindowSizeEnablesPortWindowMarginEnablesPortSynchronicityEnablesPortSignalSizeEnablesFunctionDeclFunctionTemplateSpecKindFunctionTemplateParamNamesFunctionTemplateParamKindsFunctionTemplateParamTypesFunctionTemplateParamValuesFunctionTemplateParamEnablesClassDeclClassTemplateSpecKindClassTemplateParamNamesClassTemplateParamKindsClassTemplateParamTypesClassTemplateParamValuesClassTemplateParamEnablesClassCtorDeclsClassCtorParamNamesClassCtorParamTypesClassCtorParamSerializedTypes[1 1]@C[28 1]@t6@filtert42@../../../src/aie_kernels/FirSingleStream.hC[3 1]@t3@sint3@cint4@soutC[3 1]@t21@input_stream_cint16 *t26@input_stream< cacc48_t > *t22@output_stream_cint16 *C[3 1]@t33@{P{Tinput_stream{1{t{Scint16}}}}}t35@{P{Tinput_stream{1{t{Scacc48_t}}}}}t34@{P{Toutput_stream{1{t{Scint16}}}}}C[3 1]@t5@inputt5@inputt6@outputC[3 1]@l0@l0@l0@C[3 1]@l0@l0@l0@C[3 1]@l0@l0@l0@C[3 1]@l0@l0@l1@t190@namespace SingleStream {
      | template < int NSamples, int ShiftAcc > 
      | void FIR_MultiKernel_cin::
      | filter(input_stream_cint16 * sin, input_stream< cacc48_t > * cin, output_stream_cint16 * sout);
      | }t4@nonee[0 1]@e[0 1]@e[0 1]@e[0 1]@e[0 1]@t93@namespace SingleStream {
      | template < int NSamples, int ShiftAcc > class FIR_MultiKernel_cin;
      | }t8@implicitC[2 1]@t8@NSamplest8@ShiftAccC[2 1]@t7@nontypet7@nontypeC[2 1]@t3@intt3@intC[2 1]@nnC[2 1]@l1@l1@C[1 1]@t69@FIR_MultiKernel_cin(cint16 const ( & taps ) [ 8 ], int32 const Delay)C[1 1]@C[2 1]@t4@tapst5@DelayC[1 1]@C[2 1]@t23@cint16 const ( &) [ 8 ]t11@int32 constC[1 1]@C[2 1]@t20@{R{Q1{C{Scint16}8}}}t10@{Q1{Bi32}}
      FunctionDecl=|
      | namespace SingleStream {
      | template < int NSamples, int ShiftAcc > 
      | void FIR_MultiKernel_cin::
      | filter(input_stream_cint16 * sin, input_stream< cacc48_t > * cin, output_stream_cint16 * sout);
      | }
      ClassDeclTypeOptions=|
      | C[1 1]@t93@namespace SingleStream {
      | template < int NSamples, int ShiftAcc > class FIR_MultiKernel_cin;
      | }
      ClassDecl=|
      | namespace SingleStream {
      | template < int NSamples, int ShiftAcc > class FIR_MultiKernel_cin;
      | }
  AIE Class Kernel9 : ModelComposer/AIE Class Kernel  KernelAllAttrs=|  PortNames={'sin'; 'cout'}  PortSerializedTypes={'{P{Tinput_stream{1{t{Scint16}}}}}'; '{P{Toutput_stream{1{t{Scacc48_t}}}}}'}  PortWindowSizes={0.000000000000000000e+00; 0.000000000000000000e+00}  PortWindowMargins={0.000000000000000000e+00; 0.000000000000000000e+00}  PortSynchronicities={'auto'; 'auto'}  PortSignalSizes={0.000000000000000000e+00; 4.000000000000000000e+00}  ClassTemplateSpecKind=implicit  ClassTemplateParamNames={'NSamples'; 'ShiftAcc'}  ClassTemplateParamKinds={'nontype'; 'nontype'}  ClassTemplateParamTypes={'int'; 'int'}  ClassTemplateParamValues={'512', '15'}  ClassCtorParamNames={'taps'; 'Delay'}  ClassCtorParamSerializedTypes={'{R{Q1{C{Scint16}8}}}'; '{Q1{Bi32}}'}  ClassCtorParamValues={'[-21+26i 146-91i 1183+239i 4086+5221i 248-2878i 237-54i -160+111i -83-21i]', '1'}  ClassIndex=1  ClassCtorIndex=1  ClassTabVisible=on  ClassTemplateParamsVisible=on  ClassCtorDeclVisible=on  ClassCtorParamsVisible=on  FunctionTabVisible=on  FunctionDecl=|  PortAttrs={ 'input', 'sin', 'input_stream_cint16 *', '', '', '', ''; 'output', 'cout', 'output_stream< cacc48_t > *', '', '', '', 'N' }  PortAttrsEnables={'off', 'off', 'off', 'off', 'off', 'off', 'off';'off', 'off', 'off', 'off', 'off', 'off', 'on'}  SampleTime=-1  ClassDeclTypeOptions=|  ClassDecl=|  ClassTemplateParams={ 'NSamples', 'int', 'BURST_LENGTH'; 'ShiftAcc', 'int', 'SHIFT_ACC' }  ClassTemplateParamsEnables={'off', 'off', 'on';'off', 'off', 'on'}  ClassCtorDeclTypeOptions=C[1 1]@t70@FIR_MultiKernel_cout(cint16 const ( & taps ) [ 8 ], int32 const Delay)  ClassCtorDecl=FIR_MultiKernel_cout(cint16 const ( & taps ) [ 8 ], int32 const Delay)  ClassCtorParams={ 'taps', 'cint16 const ( &) [ 8 ]', 'phi_2'; 'Delay', 'int32 const', '1' }  KernelHeaderFile=FirSingleStream.h  KernelClassName=SingleStream::FIR_MultiKernel_cout  KernelFunction=filter  KernelSourceFile=FirSingleStream.cpp  KernelSearchPaths={'$SRC', '$SRC/aie_kernels'}  PreProcOptions={}  CoreRuntimeRatio=0.9  KernelLocSpec=on  ColRowLocation=LOCATION_2_0  blockJsonConstraints="[{\"type\":\"constraint\",\"constraintType\":\"coreUtilization\",\"sid\":\"341\",\"lhs\":{\"type\":\"runtimeRatio\",\"args\":{\"type\":\"kernel\",\"name\":\"SingleStreamSSR/SSR4/AIE Class Kernel9\",\"sid\":\"341\"}},\"rhs\":{\"type\":\"evaluable\",\"expr\":\"0.9\",\"value\":0.9},\"equality\":true},{\"type\":\"constraint\",\"constraintType\":\"location_kernel\",\"sid\":\"341\",\"lhs\":{\"type\":\"location\",\"templParam\":\"kernel\",\"args\":{\"type\":\"kernel\",\"name\":\"SingleStreamSSR/SSR4/AIE Class Kernel9\",\"sid\":\"341\"}},\"rhs\":{\"type\":\"tile\",\"args\":[{\"type\":\"evaluable\",\"expr\":\"25\",\"value\":25},{\"type\":\"evaluable\",\"expr\":\"2\",\"value\":2}]},\"equality\":true}]"  deprecateConstraints=1
      KernelAllAttrs=|
      | s[12;12;9;9;19;14;21;23;24;21;12;24;26;26;26;27;28;9;21;23;23;23;24;25;14;19;19;29]@FunctionNameDeclFileNamePortNamesPortTypesPortSerializedTypesPortDirectionsPortWindowSizeEnablesPortWindowMarginEnablesPortSynchronicityEnablesPortSignalSizeEnablesFunctionDeclFunctionTemplateSpecKindFunctionTemplateParamNamesFunctionTemplateParamKindsFunctionTemplateParamTypesFunctionTemplateParamValuesFunctionTemplateParamEnablesClassDeclClassTemplateSpecKindClassTemplateParamNamesClassTemplateParamKindsClassTemplateParamTypesClassTemplateParamValuesClassTemplateParamEnablesClassCtorDeclsClassCtorParamNamesClassCtorParamTypesClassCtorParamSerializedTypes[1 1]@C[28 1]@t6@filtert42@../../../src/aie_kernels/FirSingleStream.hC[2 1]@t3@sint4@coutC[2 1]@t21@input_stream_cint16 *t27@output_stream< cacc48_t > *C[2 1]@t33@{P{Tinput_stream{1{t{Scint16}}}}}t36@{P{Toutput_stream{1{t{Scacc48_t}}}}}C[2 1]@t5@inputt6@outputC[2 1]@l0@l0@C[2 1]@l0@l0@C[2 1]@l0@l0@C[2 1]@l0@l1@t164@namespace SingleStream {
      | template < int NSamples, int ShiftAcc > 
      | void FIR_MultiKernel_cout::
      | filter(input_stream_cint16 * sin, output_stream< cacc48_t > * cout);
      | }t4@nonee[0 1]@e[0 1]@e[0 1]@e[0 1]@e[0 1]@t94@namespace SingleStream {
      | template < int NSamples, int ShiftAcc > class FIR_MultiKernel_cout;
      | }t8@implicitC[2 1]@t8@NSamplest8@ShiftAccC[2 1]@t7@nontypet7@nontypeC[2 1]@t3@intt3@intC[2 1]@nnC[2 1]@l1@l1@C[1 1]@t70@FIR_MultiKernel_cout(cint16 const ( & taps ) [ 8 ], int32 const Delay)C[1 1]@C[2 1]@t4@tapst5@DelayC[1 1]@C[2 1]@t23@cint16 const ( &) [ 8 ]t11@int32 constC[1 1]@C[2 1]@t20@{R{Q1{C{Scint16}8}}}t10@{Q1{Bi32}}
      FunctionDecl=|
      | namespace SingleStream {
      | template < int NSamples, int ShiftAcc > 
      | void FIR_MultiKernel_cout::
      | filter(input_stream_cint16 * sin, output_stream< cacc48_t > * cout);
      | }
      ClassDeclTypeOptions=|
      | C[1 1]@t94@namespace SingleStream {
      | template < int NSamples, int ShiftAcc > class FIR_MultiKernel_cout;
      | }
      ClassDecl=|
      | namespace SingleStream {
      | template < int NSamples, int ShiftAcc > class FIR_MultiKernel_cout;
      | }
  AIE Signal Spec{,1..11} (12 alike) : ModelComposer/AIE Signal Spec  FifoDepth=0  PlioWidth=64  PlioFreqSpec=on  PlioFreq=PLIO_FREQ
  PhaseOut0 : Outport
  PhaseOut1 : Outport  Port=2
  PhaseOut2 : Outport  Port=3
  PhaseOut3 : Outport  Port=4
  wires:
  AIE Class Kernel7/1 -> AIE Class Kernel8/2
  AIE Class Kernel4/1 -> AIE Class Kernel13/2
  AIE Class Kernel5/1 -> AIE Class Kernel10/2
  AIE Class Kernel15/1 -> AIE Class Kernel16/2
  AIE Class Kernel9/1 -> AIE Class Kernel6/2
  AIE Class Kernel12/1 -> AIE Class Kernel5/2
  AIE Class Kernel13/1 -> AIE Class Kernel15/2
  AIE Class Kernel1/1 -> AIE Class Kernel11/2
  AIE Class Kernel11/1 -> AIE Class Kernel3/2
  AIE Class Kernel6/1 -> AIE Class Kernel7/2
  AIE Class Kernel10/1 -> AIE Class Kernel17/2
  AIE Class Kernel3/1 -> AIE Class Kernel18/2
  AIE Class Kernel16/1 -> AIE Signal Spec9/1
  AIE Class Kernel17/1 -> AIE Signal Spec8/1
  PhaseIn0_0/1 -> AIE Signal Spec/1
  PhaseIn0_1/1 -> AIE Signal Spec1/1
  PhaseIn1_0/1 -> AIE Signal Spec2/1
  PhaseIn1_1/1 -> AIE Signal Spec3/1
  PhaseIn2_0/1 -> AIE Signal Spec4/1
  PhaseIn2_1/1 -> AIE Signal Spec5/1
  PhaseIn3_0/1 -> AIE Signal Spec6/1
  PhaseIn3_1/1 -> AIE Signal Spec7/1
  AIE Class Kernel8/1 -> AIE Signal Spec10/1
  AIE Class Kernel18/1 -> AIE Signal Spec11/1
  AIE Signal Spec/1 -> AIE Class Kernel1/1, AIE Class Kernel9/1
  AIE Signal Spec1/1 -> AIE Class Kernel17/1, AIE Class Kernel16/1
  AIE Signal Spec2/1 -> AIE Class Kernel11/1, AIE Class Kernel6/1
  AIE Signal Spec3/1 -> AIE Class Kernel10/1, AIE Class Kernel15/1
  AIE Signal Spec4/1 -> AIE Class Kernel3/1, AIE Class Kernel7/1
  AIE Signal Spec5/1 -> AIE Class Kernel5/1, AIE Class Kernel13/1
  AIE Signal Spec6/1 -> AIE Class Kernel18/1, AIE Class Kernel8/1
  AIE Signal Spec7/1 -> AIE Class Kernel12/1, AIE Class Kernel4/1
  AIE Signal Spec8/1 -> PhaseOut1/1
  AIE Signal Spec9/1 -> PhaseOut3/1
  AIE Signal Spec10/1 -> PhaseOut2/1
  AIE Signal Spec11/1 -> PhaseOut0/1
